simulink model "COMPONENT_MDL_Lag_QUAD_and_PEND_with_spin_rotors"  (R2020b)
(part 10 of 10)

(Lx_pend.^2.*THE_Theta_D.*m_pend.*sin(THE_Theta_pend.*2.0))./2.4e+1-(Ly_pend.^2.*THE_Theta_D.*m_pend.*sin(THE_Theta_pend.*2.0))./2.4e+1-(Lx_pend.^2.*THE_Psi_D.*m_pend.*cos(THE_Phi_pend).*sin(THE_Psi))./6.0-(Ly_pend.^2.*THE_Phi_pend_D.*m_pend.*cos(THE_Psi).*sin(THE_Phi_pend))./6.0-(Ly_pend.^2.*THE_Psi_pend_D.*m_pend.*cos(THE_Theta_pend).*sin(THE_Psi))./6.0-(Lx_pend.^2.*THE_Theta_D.*m_pend.*cos(THE_Psi).*sin(THE_Psi).*sin(THE_Phi_pend))./1.2e+1-(Lx_pend.^2.*THE_Phi_pend_D.*m_pend.*cos(THE_Theta_pend).*sin(THE_Psi).*sin(THE_Theta_pend))./6.0+(Ly_pend.^2.*THE_Theta_D.*m_pend.*cos(THE_Psi).*sin(THE_Psi).*sin(THE_Phi_pend))./1.2e+1+(Ly_pend.^2.*THE_Psi_pend_D.*m_pend.*cos(THE_Psi).*sin(THE_Phi_pend).*sin(THE_Theta_pend))./6.0+(Ly_pend.^2.*THE_Phi_pend_D.*m_pend.*cos(THE_Theta_pend).*sin(THE_Psi).*sin(THE_Theta_pend))./6.0+(Lx_pend.^2.*THE_Psi_D.*m_pend.*cos(THE_Phi_pend).*cos(THE_Theta_pend).^2.*sin(THE_Psi))./6.0-(Lx_pend.^2.*THE_Theta_D.*m_pend.*cos(THE_Psi).^2.*cos(THE_Theta_pend).*sin(THE_Theta_pend))./6.0-(Lx_pend.^2.*THE_Phi_pend_D.*m_pend.*cos(THE_Psi).*cos(THE_Theta_pend).^2.*sin(THE_Phi_pend))./6.0-(Ly_pend.^2.*THE_Psi_D.*m_pend.*cos(THE_Phi_pend).*cos(THE_Theta_pend).^2.*sin(THE_Psi))./6.0+(Ly_pend.^2.*THE_Phi_pend_D.*m_pend.*cos(THE_Psi).*cos(THE_Psi_pend).^2.*sin(THE_Phi_pend))./6.0+(Ly_pend.^2.*THE_Theta_D.*m_pend.*cos(THE_Psi).^2.*cos(THE_Theta_pend).*sin(THE_Theta_pend))./6.0+(Ly_pend.^2.*THE_Phi_pend_D.*m_pend.*cos(THE_Psi).*cos(THE_Theta_pend).^2.*sin(THE_Phi_pend))./6.0+(Ly_pend.^2.*THE_Psi_pend_D.*m_pend.*cos(THE_Psi_pend).^2.*cos(THE_Theta_pend).*sin(THE_Psi))./6.0+(Ly_pend.^2.*THE_Theta_D.*m_pend.*cos(THE_Psi_pend).^2.*cos(THE_Theta_pend).*sin(THE_Theta_pend))./1.2e+1-Lz_pend.^2.*THE_Phi_pend_D.*m_pend.*cos(THE_Psi).*cos(THE_Psi_pend).^2.*sin(THE_Phi_pend).*(2.0./3.0)-Lz_pend.^2.*THE_Psi_pend_D.*m_pend.*cos(THE_Psi_pend).^2.*cos(THE_Theta_pend).*sin(THE_Psi).*(2.0./3.0)-(Lz_pend.^2.*THE_Theta_D.*m_pend.*cos(THE_Psi_pend).^2.*cos(THE_Theta_pend).*sin(THE_Theta_pend))./3.0+(Lx_pend.^2.*THE_Theta_D.*m_pend.*cos(THE_Psi).*cos(THE_Theta_pend).^2.*sin(THE_Psi).*sin(THE_Phi_pend))./6.0-(Ly_pend.^2.*THE_Theta_D.*m_pend.*cos(THE_Psi).*cos(THE_Psi_pend).^2.*sin(THE_Psi).*sin(THE_Phi_pend))./1.2e+1-(Ly_pend.^2.*THE_Theta_D.*m_pend.*cos(THE_Psi).*cos(THE_Theta_pend).^2.*sin(THE_Psi).*sin(THE_Phi_pend))./6.0-(Ly_pend.^2.*THE_Psi_pend_D.*m_pend.*cos(THE_Psi).*cos(THE_Psi_pend).^2.*sin(THE_Phi_pend).*sin(THE_Theta_pend))./6.0-(Ly_pend.^2.*THE_Phi_pend_D.*m_pend.*cos(THE_Psi_pend).^2.*cos(THE_Theta_pend).*sin(THE_Psi).*sin(THE_Theta_pend))./6.0+(Lz_pend.^2.*THE_Theta_D.*m_pend.*cos(THE_Psi).*cos(THE_Psi_pend).^2.*sin(THE_Psi).*sin(THE_Phi_pend))./3.0+Lz_pend.^2.*THE_Psi_pend_D.*m_pend.*cos(THE_Psi).*cos(THE_Psi_pend).^2.*sin(THE_Phi_pend).*sin(THE_Theta_pend).*(2.0./3.0)+Lz_pend.^2.*THE_Phi_pend_D.*m_pend.*cos(THE_Psi_pend).^2.*cos(THE_Theta_pend).*sin(THE_Psi).*sin(THE_Theta_pend).*(2.0./3.0)+(Lz_pend.*THE_Theta_D.*Tv_Z_pend.*m_pend.*cos(THE_Psi).^2.*cos(THE_Psi_pend).*sin(THE_Theta_pend))./2.0+(Lx_pend.^2.*THE_Theta_D.*m_pend.*cos(THE_Psi).^2.*cos(THE_Phi_pend).^2.*cos(THE_Theta_pend).*sin(THE_Theta_pend))./1.2e+1+(Ly_pend.^2.*THE_Psi_D.*m_pend.*cos(THE_Phi_pend).*cos(THE_Psi_pend).^2.*cos(THE_Theta_pend).^2.*sin(THE_Psi))./6.0-(Ly_pend.^2.*THE_Theta_D.*m_pend.*cos(THE_Psi).^2.*cos(THE_Phi_pend).^2.*cos(THE_Theta_pend).*sin(THE_Theta_pend))./1.2e+1-(Ly_pend.^2.*THE_Theta_D.*m_pend.*cos(THE_Psi).^2.*cos(THE_Psi_pend).^2.*cos(THE_Theta_pend).*sin(THE_Theta_pend))./6.0-(Ly_pend.^2.*THE_Phi_pend_D.*m_pend.*cos(THE_Psi).*cos(THE_Psi_pend).^2.*cos(THE_Theta_pend).^2.*sin(THE_Phi_pend))./6.0-Lz_pend.^2.*THE_Psi_D.*m_pend.*cos(THE_Phi_pend).*cos(THE_Psi_pend).^2.*cos(THE_Theta_pend).^2.*sin(THE_Psi).*(2.0./3.0)+Lz_pend.^2.*THE_Theta_D.*m_pend.*cos(THE_Psi).^2.*cos(THE_Psi_pend).^2.*cos(THE_Theta_pend).*sin(THE_Theta_pend).*(2.0./3.0)+Lz_pend.^2.*THE_Phi_pend_D.*m_pend.*cos(THE_Psi).*cos(THE_Psi_pend).^2.*cos(THE_Theta_pend).^2.*sin(THE_Phi_pend).*(2.0./3.0)+(Ly_pend.^2.*THE_Psi_pend_D.*m_pend.*cos(THE_Psi).*cos(THE_Phi_pend).*cos(THE_Psi_pend).*sin(THE_Psi_pend))./6.0-Lz_pend.^2.*THE_Psi_pend_D.*m_pend.*cos(THE_Psi).*cos(THE_Phi_pend).*cos(THE_Psi_pend).*sin(THE_Psi_pend).*(2.0./3.0)+(Ly_pend.^2.*THE_Theta_D.*m_pend.*cos(THE_Psi).*cos(THE_Psi_pend).^2.*cos(THE_Theta_pend).^2.*sin(THE_Psi).*sin(THE_Phi_pend))./6.0-Lz_pend.^2.*THE_Theta_D.*m_pend.*cos(THE_Psi).*cos(THE_Psi_pend).^2.*cos(THE_Theta_pend).^2.*sin(THE_Psi).*sin(THE_Phi_pend).*(2.0./3.0)-(Lx_pend.^2.*THE_Psi_D.*m_pend.*cos(THE_Psi).*cos(THE_Phi_pend).*cos(THE_Theta_pend).*sin(THE_Phi_pend).*sin(THE_Theta_pend))./6.0+(Ly_pend.^2.*THE_Psi_D.*m_pend.*cos(THE_Psi).*cos(THE_Phi_pend).*cos(THE_Theta_pend).*sin(THE_Phi_pend).*sin(THE_Theta_pend))./6.0-(Ly_pend.^2.*THE_Phi_pend_D.*m_pend.*cos(THE_Psi).*cos(THE_Phi_pend).*cos(THE_Psi_pend).*sin(THE_Psi_pend).*sin(THE_Theta_pend))./6.0+Lz_pend.^2.*THE_Phi_pend_D.*m_pend.*cos(THE_Psi).*cos(THE_Phi_pend).*cos(THE_Psi_pend).*sin(THE_Psi_pend).*sin(THE_Theta_pend).*(2.0./3.0)+(Ly_pend.^2.*THE_Theta_D.*m_pend.*cos(THE_Psi).^2.*cos(THE_Phi_pend).^2.*cos(THE_Psi_pend).^2.*cos(THE_Theta_pend).*sin(THE_Theta_pend))./1.2e+1-(Lz_pend.^2.*THE_Theta_D.*m_pend.*cos(THE_Psi).^2.*cos(THE_Phi_pend).^2.*cos(THE_Psi_pend).^2.*cos(THE_Theta_pend).*sin(THE_Theta_pend))./3.0-Lz_pend.*THE_Psi_D.*Tv_Z_pend.*m_pend.*cos(THE_Phi_pend).*cos(THE_Psi_pend).*cos(THE_Theta_pend).*sin(THE_Psi)+(Ly_pend.^2.*THE_Psi_D.*m_pend.*cos(THE_Psi).*cos(THE_Phi_pend).^2.*cos(THE_Psi_pend).*cos(THE_Theta_pend).*sin(THE_Psi_pend))./6.0-Lz_pend.^2.*THE_Psi_D.*m_pend.*cos(THE_Psi).*cos(THE_Phi_pend).^2.*cos(THE_Psi_pend).*cos(THE_Theta_pend).*sin(THE_Psi_pend).*(2.0./3.0)+(Ly_pend.^2.*THE_Theta_D.*m_pend.*cos(THE_Psi).*cos(THE_Phi_pend).*cos(THE_Psi_pend).*sin(THE_Psi).*sin(THE_Psi_pend).*sin(THE_Theta_pend))./1.2e+1-(Lz_pend.^2.*THE_Theta_D.*m_pend.*cos(THE_Psi).*cos(THE_Phi_pend).*cos(THE_Psi_pend).*sin(THE_Psi).*sin(THE_Psi_pend).*sin(THE_Theta_pend))./3.0-(Lz_pend.*THE_Theta_D.*Tv_Z_pend.*m_pend.*cos(THE_Psi).*cos(THE_Psi_pend).*cos(THE_Theta_pend).*sin(THE_Psi).*sin(THE_Phi_pend))./2.0-(Ly_pend.^2.*THE_Psi_D.*m_pend.*cos(THE_Psi).*cos(THE_Phi_pend).*cos(THE_Psi_pend).^2.*cos(THE_Theta_pend).*sin(THE_Phi_pend).*sin(THE_Theta_pend))./6.0+(Ly_pend.^2.*THE_Theta_D.*m_pend.*cos(THE_Psi).^2.*cos(THE_Phi_pend).*cos(THE_Psi_pend).*cos(THE_Theta_pend).*sin(THE_Phi_pend).*sin(THE_Psi_pend))./1.2e+1+Lz_pend.^2.*THE_Psi_D.*m_pend.*cos(THE_Psi).*cos(THE_Phi_pend).*cos(THE_Psi_pend).^2.*cos(THE_Theta_pend).*sin(THE_Phi_pend).*sin(THE_Theta_pend).*(2.0./3.0)-(Lz_pend.^2.*THE_Theta_D.*m_pend.*cos(THE_Psi).^2.*cos(THE_Phi_pend).*cos(THE_Psi_pend).*cos(THE_Theta_pend).*sin(THE_Phi_pend).*sin(THE_Psi_pend))./3.0,(Ly_pend.^2.*THE_Psi_D.*m_pend.*cos(THE_Psi).*sin(THE_Theta_pend))./6.0+(Ly_pend.^2.*THE_Theta_pend_D.*m_pend.*cos(THE_Theta_pend).*sin(THE_Psi))./6.0-(Ly_pend.^2.*THE_Psi_D.*m_pend.*cos(THE_Theta_pend).*sin(THE_Psi).*sin(THE_Phi_pend))./6.0-(Ly_pend.^2.*THE_Theta_pend_D.*m_pend.*cos(THE_Psi).*sin(THE_Phi_pend).*sin(THE_Theta_pend))./6.0-(Ly_pend.^2.*THE_Psi_D.*m_pend.*cos(THE_Psi).*cos(THE_Phi_pend).^2.*sin(THE_Theta_pend))./6.0-(Ly_pend.^2.*THE_Psi_D.*m_pend.*cos(THE_Psi).*cos(THE_Psi_pend).^2.*sin(THE_Theta_pend))./6.0+(Ly_pend.^2.*THE_Theta_D.*m_pend.*cos(THE_Psi).^2.*cos(THE_Psi_pend).*sin(THE_Psi_pend))./1.2e+1+(Ly_pend.^2.*THE_Theta_D.*m_pend.*cos(THE_Psi_pend).*cos(THE_Theta_pend).^2.*sin(THE_Psi_pend))./1.2e+1-(Ly_pend.^2.*THE_Theta_pend_D.*m_pend.*cos(THE_Psi_pend).^2.*cos(THE_Theta_pend).*sin(THE_Psi))./6.0+Lz_pend.^2.*THE_Psi_D.*m_pend.*cos(THE_Psi).*cos(THE_Phi_pend).^2.*sin(THE_Theta_pend).*(2.0./3.0)+Lz_pend.^2.*THE_Psi_D.*m_pend.*cos(THE_Psi).*cos(THE_Psi_pend).^2.*sin(THE_Theta_pend).*(2.0./3.0)-(Lz_pend.^2.*THE_Theta_D.*m_pend.*cos(THE_Psi).^2.*cos(THE_Psi_pend).*sin(THE_Psi_pend))./3.0-(Lz_pend.^2.*THE_Theta_D.*m_pend.*cos(THE_Psi_pend).*cos(THE_Theta_pend).^2.*sin(THE_Psi_pend))./3.0+Lz_pend.^2.*THE_Theta_pend_D.*m_pend.*cos(THE_Psi_pend).^2.*cos(THE_Theta_pend).*sin(THE_Psi).*(2.0./3.0)+Lz_pend.^2.*THE_Phi_pend_D.*m_pend.*cos(THE_Psi).*cos(THE_Phi_pend).*cos(THE_Theta_pend).*(2.0./3.0)-Lz_pend.*THE_Psi_D.*Tv_Z_pend.*m_pend.*cos(THE_Psi_pend).*sin(THE_Psi).*sin(THE_Phi_pend)+(Ly_pend.^2.*THE_Phi_pend_D.*m_pend.*cos(THE_Psi).*cos(THE_Phi_pend).*cos(THE_Psi_pend).^2.*cos(THE_Theta_pend))./6.0-Lz_pend.^2.*THE_Phi_pend_D.*m_pend.*cos(THE_Psi).*cos(THE_Phi_pend).*cos(THE_Psi_pend).^2.*cos(THE_Theta_pend).*(2.0./3.0)+(Ly_pend.^2.*THE_Psi_D.*m_pend.*cos(THE_Psi_pend).^2.*cos(THE_Theta_pend).*sin(THE_Psi).*sin(THE_Phi_pend))./6.0-(Ly_pend.^2.*THE_Theta_D.*m_pend.*cos(THE_Psi).^2.*cos(THE_Phi_pend).*sin(THE_Phi_pend).*sin(THE_Theta_pend))./1.2e+1-(Ly_pend.^2.*THE_Phi_pend_D.*m_pend.*cos(THE_Psi_pend).*cos(THE_Theta_pend).^2.*sin(THE_Psi).*sin(THE_Psi_pend))./6.0+(Ly_pend.^2.*THE_Theta_pend_D.*m_pend.*cos(THE_Psi).*cos(THE_Psi_pend).^2.*sin(THE_Phi_pend).*sin(THE_Theta_pend))./6.0-Lz_pend.^2.*THE_Psi_D.*m_pend.*cos(THE_Psi_pend).^2.*cos(THE_Theta_pend).*sin(THE_Psi).*sin(THE_Phi_pend).*(2.0./3.0)+(Lz_pend.^2.*THE_Theta_D.*m_pend.*cos(THE_Psi).^2.*cos(THE_Phi_pend).*sin(THE_Phi_pend).*sin(THE_Theta_pend))./3.0+Lz_pend.^2.*THE_Phi_pend_D.*m_pend.*cos(THE_Psi_pend).*cos(THE_Theta_pend).^2.*sin(THE_Psi).*sin(THE_Psi_pend).*(2.0./3.0)-Lz_pend.^2.*THE_Theta_pend_D.*m_pend.*cos(THE_Psi).*cos(THE_Psi_pend).^2.*sin(THE_Phi_pend).*sin(THE_Theta_pend).*(2.0./3.0)+(Lz_pend.*THE_Theta_D.*Tv_Z_pend.*m_pend.*cos(THE_Psi).^2.*cos(THE_Theta_pend).*sin(THE_Psi_pend))./2.0+(Ly_pend.^2.*THE_Psi_D.*m_pend.*cos(THE_Psi).*cos(THE_Phi_pend).^2.*cos(THE_Psi_pend).^2.*sin(THE_Theta_pend))./3.0-(Ly_pend.^2.*THE_Theta_D.*m_pend.*cos(THE_Psi).^2.*cos(THE_Phi_pend).^2.*cos(THE_Psi_pend).*sin(THE_Psi_pend))./6.0-(Ly_pend.^2.*THE_Theta_D.*m_pend.*cos(THE_Psi).^2.*cos(THE_Psi_pend).*cos(THE_Theta_pend).^2.*sin(THE_Psi_pend))./6.0-Lz_pend.^2.*THE_Psi_D.*m_pend.*cos(THE_Psi).*cos(THE_Phi_pend).^2.*cos(THE_Psi_pend).^2.*sin(THE_Theta_pend).*(4.0./3.0)+Lz_pend.^2.*THE_Theta_D.*m_pend.*cos(THE_Psi).^2.*cos(THE_Phi_pend).^2.*cos(THE_Psi_pend).*sin(THE_Psi_pend).*(2.0./3.0)+Lz_pend.^2.*THE_Theta_D.*m_pend.*cos(THE_Psi).^2.*cos(THE_Psi_pend).*cos(THE_Theta_pend).^2.*sin(THE_Psi_pend).*(2.0./3.0)+(Ly_pend.^2.*THE_Theta_D.*m_pend.*cos(THE_Psi).*cos(THE_Phi_pend).*cos(THE_Theta_pend).*sin(THE_Psi))./1.2e+1-(Ly_pend.^2.*THE_Theta_pend_D.*m_pend.*cos(THE_Psi).*cos(THE_Phi_pend).*cos(THE_Psi_pend).*sin(THE_Psi_pend))./6.0-(Lz_pend.^2.*THE_Theta_D.*m_pend.*cos(THE_Psi).*cos(THE_Phi_pend).*cos(THE_Theta_pend).*sin(THE_Psi))./3.0+Lz_pend.^2.*THE_Theta_pend_D.*m_pend.*cos(THE_Psi).*cos(THE_Phi_pend).*cos(THE_Psi_pend).*sin(THE_Psi_pend).*(2.0./3.0)+(Ly_pend.^2.*THE_Theta_D.*m_pend.*cos(THE_Psi).^2.*cos(THE_Phi_pend).*cos(THE_Psi_pend).^2.*sin(THE_Phi_pend).*sin(THE_Theta_pend))./6.0-Lz_pend.^2.*THE_Theta_D.*m_pend.*cos(THE_Psi).^2.*cos(THE_Phi_pend).*cos(THE_Psi_pend).^2.*sin(THE_Phi_pend).*sin(THE_Theta_pend).*(2.0./3.0)+(Ly_pend.^2.*THE_Psi_D.*m_pend.*cos(THE_Psi).*cos(THE_Phi_pend).*cos(THE_Psi_pend).*sin(THE_Phi_pend).*sin(THE_Psi_pend))./3.0-Lz_pend.^2.*THE_Psi_D.*m_pend.*cos(THE_Psi).*cos(THE_Phi_pend).*cos(THE_Psi_pend).*sin(THE_Phi_pend).*sin(THE_Psi_pend).*(4.0./3.0)+(Ly_pend.^2.*THE_Theta_D.*m_pend.*cos(THE_Psi).^2.*cos(THE_Phi_pend).^2.*cos(THE_Psi_pend).*cos(THE_Theta_pend).^2.*sin(THE_Psi_pend))./1.2e+1-(Lz_pend.^2.*THE_Theta_D.*m_pend.*cos(THE_Psi).^2.*cos(THE_Phi_pend).^2.*cos(THE_Psi_pend).*cos(THE_Theta_pend).^2.*sin(THE_Psi_pend))./3.0+(Lz_pend.*THE_Theta_D.*Tv_Z_pend.*m_pend.*cos(THE_Psi).*cos(THE_Phi_pend).*cos(THE_Psi_pend).*sin(THE_Psi))./2.0+Lz_pend.*THE_Psi_D.*Tv_Z_pend.*m_pend.*cos(THE_Phi_pend).*sin(THE_Psi).*sin(THE_Psi_pend).*sin(THE_Theta_pend)-(Ly_pend.^2.*THE_Theta_D.*m_pend.*cos(THE_Psi).*cos(THE_Phi_pend).*cos(THE_Psi_pend).^2.*cos(THE_Theta_pend).*sin(THE_Psi))./6.0+Lz_pend.^2.*THE_Theta_D.*m_pend.*cos(THE_Psi).*cos(THE_Phi_pend).*cos(THE_Psi_pend).^2.*cos(THE_Theta_pend).*sin(THE_Psi).*(2.0./3.0)-(Ly_pend.^2.*THE_Psi_D.*m_pend.*cos(THE_Phi_pend).*cos(THE_Psi_pend).*cos(THE_Theta_pend).*sin(THE_Psi).*sin(THE_Psi_pend).*sin(THE_Theta_pend))./6.0+(Ly_pend.^2.*THE_Phi_pend_D.*m_pend.*cos(THE_Psi).*cos(THE_Psi_pend).*cos(THE_Theta_pend).*sin(THE_Phi_pend).*sin(THE_Psi_pend).*sin(THE_Theta_pend))./6.0+Lz_pend.^2.*THE_Psi_D.*m_pend.*cos(THE_Phi_pend).*cos(THE_Psi_pend).*cos(THE_Theta_pend).*sin(THE_Psi).*sin(THE_Psi_pend).*sin(THE_Theta_pend).*(2.0./3.0)-Lz_pend.^2.*THE_Phi_pend_D.*m_pend.*cos(THE_Psi).*cos(THE_Psi_pend).*cos(THE_Theta_pend).*sin(THE_Phi_pend).*sin(THE_Psi_pend).*sin(THE_Theta_pend).*(2.0./3.0)+(Lz_pend.*THE_Theta_D.*Tv_Z_pend.*m_pend.*cos(THE_Psi).*sin(THE_Psi).*sin(THE_Phi_pend).*sin(THE_Psi_pend).*sin(THE_Theta_pend))./2.0-(Ly_pend.^2.*THE_Psi_D.*m_pend.*cos(THE_Psi).*cos(THE_Phi_pend).*cos(THE_Psi_pend).*cos(THE_Theta_pend).^2.*sin(THE_Phi_pend).*sin(THE_Psi_pend))./6.0+Lz_pend.^2.*THE_Psi_D.*m_pend.*cos(THE_Psi).*cos(THE_Phi_pend).*cos(THE_Psi_pend).*cos(THE_Theta_pend).^2.*sin(THE_Phi_pend).*sin(THE_Psi_pend).*(2.0./3.0)-(Ly_pend.^2.*THE_Theta_D.*m_pend.*cos(THE_Psi).*cos(THE_Psi_pend).*cos(THE_Theta_pend).*sin(THE_Psi).*sin(THE_Phi_pend).*sin(THE_Psi_pend).*sin(THE_Theta_pend))./6.0+Lz_pend.^2.*THE_Theta_D.*m_pend.*cos(THE_Psi).*cos(THE_Psi_pend).*cos(THE_Theta_pend).*sin(THE_Psi).*sin(THE_Phi_pend).*sin(THE_Psi_pend).*sin(THE_Theta_pend).*(2.0./3.0),I_xy.*THE_Psi_D.*cos(THE_Psi).*cos(THE_Theta)+Iprop_xy.*THE_Psi_D.*cos(THE_Psi).*cos(THE_Theta).*4.0-I_xz.*THE_Psi_D.*cos(THE_Theta).*sin(THE_Psi)-Iprop_xz.*THE_Psi_D.*cos(THE_Theta).*sin(THE_Psi).*4.0+Iprop_yz.*wMOT_1.*cos(THE_Psi).*cos(THE_Theta)+Iprop_yz.*wMOT_2.*cos(THE_Psi).*cos(THE_Theta)+Iprop_yz.*wMOT_3.*cos(THE_Psi).*cos(THE_Theta)+Iprop_yz.*wMOT_4.*cos(THE_Psi).*cos(THE_Theta)-Iprop_zz.*wMOT_1.*cos(THE_Theta).*sin(THE_Psi)-Iprop_zz.*wMOT_2.*cos(THE_Theta).*sin(THE_Psi)-Iprop_zz.*wMOT_3.*cos(THE_Theta).*sin(THE_Psi)-Iprop_zz.*wMOT_4.*cos(THE_Theta).*sin(THE_Psi)-Lz_pend.^2.*THE_Phi_pend_D.*m_pend.*cos(THE_Theta).*sin(THE_Psi).*(2.0./3.0)-(Ly_pend.^2.*THE_Phi_pend_D.*m_pend.*cos(THE_Phi_pend).*sin(THE_Theta).*sin(THE_Phi_pend))./6.0-(Ly_pend.^2.*THE_Psi_pend_D.*m_pend.*cos(THE_Psi_pend).*sin(THE_Theta).*sin(THE_Psi_pend))./6.0+Lz_pend.^2.*THE_Psi_pend_D.*m_pend.*cos(THE_Theta).*sin(THE_Psi).*sin(THE_Theta_pend).*(2.0./3.0)+Lz_pend.^2.*THE_Phi_pend_D.*m_pend.*cos(THE_Phi_pend).*sin(THE_Theta).*sin(THE_Phi_pend).*(2.0./3.0)+Lz_pend.^2.*THE_Psi_pend_D.*m_pend.*cos(THE_Psi_pend).*sin(THE_Theta).*sin(THE_Psi_pend).*(2.0./3.0)-(Ly_pend.^2.*THE_Phi_pend_D.*m_pend.*cos(THE_Theta).*cos(THE_Phi_pend).^2.*sin(THE_Psi))./6.0-(Ly_pend.^2.*THE_Phi_pend_D.*m_pend.*cos(THE_Theta).*cos(THE_Psi_pend).^2.*sin(THE_Psi))./6.0+Lz_pend.^2.*THE_Phi_pend_D.*m_pend.*cos(THE_Theta).*cos(THE_Phi_pend).^2.*sin(THE_Psi).*(2.0./3.0)+Lz_pend.^2.*THE_Phi_pend_D.*m_pend.*cos(THE_Theta).*cos(THE_Psi_pend).^2.*sin(THE_Psi).*(2.0./3.0)+(Ly_pend.^2.*THE_Theta_pend_D.*m_pend.*cos(THE_Psi).*cos(THE_Theta).*cos(THE_Phi_pend))./6.0+Lz_pend.*THE_Psi_pend_D.*Tv_Z_pend.*m_pend.*cos(THE_Theta_pend).*sin(THE_Theta).*sin(THE_Psi_pend)+Lz_pend.*THE_Theta_pend_D.*Tv_Z_pend.*m_pend.*cos(THE_Psi_pend).*sin(THE_Theta).*sin(THE_Theta_pend)+(Lx_pend.^2.*THE_Theta_pend_D.*m_pend.*cos(THE_Psi).*cos(THE_Theta).*cos(THE_Phi_pend).*cos(THE_Theta_pend).^2)./6.0-(Ly_pend.^2.*THE_Theta_pend_D.*m_pend.*cos(THE_Psi).*cos(THE_Theta).*cos(THE_Phi_pend).*cos(THE_Psi_pend).^2)./6.0-(Ly_pend.^2.*THE_Theta_pend_D.*m_pend.*cos(THE_Psi).*cos(THE_Theta).*cos(THE_Phi_pend).*cos(THE_Theta_pend).^2)./6.0+Lz_pend.^2.*THE_Theta_pend_D.*m_pend.*cos(THE_Psi).*cos(THE_Theta).*cos(THE_Phi_pend).*cos(THE_Psi_pend).^2.*(2.0./3.0)-(Lx_pend.^2.*THE_Phi_pend_D.*m_pend.*cos(THE_Phi_pend).*cos(THE_Theta_pend).^2.*sin(THE_Theta).*sin(THE_Phi_pend))./6.0-(Lx_pend.^2.*THE_Theta_pend_D.*m_pend.*cos(THE_Phi_pend).^2.*cos(THE_Theta_pend).*sin(THE_Theta).*sin(THE_Theta_pend))./6.0+(Ly_pend.^2.*THE_Psi_pend_D.*m_pend.*cos(THE_Theta).*cos(THE_Phi_pend).^2.*sin(THE_Psi).*sin(THE_Theta_pend))./6.0+(Ly_pend.^2.*THE_Psi_pend_D.*m_pend.*cos(THE_Theta).*cos(THE_Psi_pend).^2.*sin(THE_Psi).*sin(THE_Theta_pend))./6.0+(Ly_pend.^2.*THE_Phi_pend_D.*m_pend.*cos(THE_Phi_pend).*cos(THE_Psi_pend).^2.*sin(THE_Theta).*sin(THE_Phi_pend))./3.0+(Ly_pend.^2.*THE_Psi_pend_D.*m_pend.*cos(THE_Phi_pend).^2.*cos(THE_Psi_pend).*sin(THE_Theta).*sin(THE_Psi_pend))./3.0+(Ly_pend.^2.*THE_Phi_pend_D.*m_pend.*cos(THE_Phi_pend).*cos(THE_Theta_pend).^2.*sin(THE_Theta).*sin(THE_Phi_pend))./6.0+(Ly_pend.^2.*THE_Theta_pend_D.*m_pend.*cos(THE_Phi_pend).^2.*cos(THE_Theta_pend).*sin(THE_Theta).*sin(THE_Theta_pend))./6.0-Lz_pend.^2.*THE_Psi_pend_D.*m_pend.*cos(THE_Theta).*cos(THE_Phi_pend).^2.*sin(THE_Psi).*sin(THE_Theta_pend).*(2.0./3.0)-Lz_pend.^2.*THE_Psi_pend_D.*m_pend.*cos(THE_Theta).*cos(THE_Psi_pend).^2.*sin(THE_Psi).*sin(THE_Theta_pend).*(2.0./3.0)-Lz_pend.^2.*THE_Phi_pend_D.*m_pend.*cos(THE_Phi_pend).*cos(THE_Psi_pend).^2.*sin(THE_Theta).*sin(THE_Phi_pend).*(4.0./3.0)-Lz_pend.^2.*THE_Psi_pend_D.*m_pend.*cos(THE_Phi_pend).^2.*cos(THE_Psi_pend).*sin(THE_Theta).*sin(THE_Psi_pend).*(4.0./3.0)-(Lx_pend.^2.*THE_Phi_pend_D.*m_pend.*cos(THE_Theta).*cos(THE_Phi_pend).^2.*cos(THE_Theta_pend).^2.*sin(THE_Psi))./6.0+(Ly_pend.^2.*THE_Phi_pend_D.*m_pend.*cos(THE_Theta).*cos(THE_Phi_pend).^2.*cos(THE_Psi_pend).^2.*sin(THE_Psi))./3.0+(Ly_pend.^2.*THE_Phi_pend_D.*m_pend.*cos(THE_Theta).*cos(THE_Phi_pend).^2.*cos(THE_Theta_pend).^2.*sin(THE_Psi))./6.0-Lz_pend.^2.*THE_Phi_pend_D.*m_pend.*cos(THE_Theta).*cos(THE_Phi_pend).^2.*cos(THE_Psi_pend).^2.*sin(THE_Psi).*(4.0./3.0)-(Ly_pend.^2.*THE_Psi_D.*m_pend.*cos(THE_Psi).*cos(THE_Theta).*cos(THE_Phi_pend).*sin(THE_Phi_pend))./1.2e+1+(Lz_pend.^2.*THE_Psi_D.*m_pend.*cos(THE_Psi).*cos(THE_Theta).*cos(THE_Phi_pend).*sin(THE_Phi_pend))./3.0+Lz_pend.^2.*THE_Psi_pend_D.*m_pend.*cos(THE_Psi).*cos(THE_Theta).*cos(THE_Theta_pend).*sin(THE_Phi_pend).*(2.0./3.0)+(Ly_pend.^2.*THE_Psi_pend_D.*m_pend.*cos(THE_Phi_pend).*sin(THE_Theta).*sin(THE_Phi_pend).*sin(THE_Theta_pend))./6.0+(Ly_pend.^2.*THE_Phi_pend_D.*m_pend.*cos(THE_Psi_pend).*sin(THE_Theta).*sin(THE_Psi_pend).*sin(THE_Theta_pend))./6.0-Lz_pend.^2.*THE_Psi_pend_D.*m_pend.*cos(THE_Phi_pend).*sin(THE_Theta).*sin(THE_Phi_pend).*sin(THE_Theta_pend).*(2.0./3.0)-Lz_pend.^2.*THE_Phi_pend_D.*m_pend.*cos(THE_Psi_pend).*sin(THE_Theta).*sin(THE_Psi_pend).*sin(THE_Theta_pend).*(2.0./3.0)+(Ly_pend.^2.*THE_Theta_pend_D.*m_pend.*cos(THE_Psi).*cos(THE_Theta).*cos(THE_Phi_pend).*cos(THE_Psi_pend).^2.*cos(THE_Theta_pend).^2)./6.0-Lz_pend.^2.*THE_Theta_pend_D.*m_pend.*cos(THE_Psi).*cos(THE_Theta).*cos(THE_Phi_pend).*cos(THE_Psi_pend).^2.*cos(THE_Theta_pend).^2.*(2.0./3.0)-(Ly_pend.^2.*THE_Psi_pend_D.*m_pend.*cos(THE_Theta).*cos(THE_Phi_pend).^2.*cos(THE_Psi_pend).^2.*sin(THE_Psi).*sin(THE_Theta_pend))./3.0-(Ly_pend.^2.*THE_Phi_pend_D.*m_pend.*cos(THE_Phi_pend).*cos(THE_Psi_pend).^2.*cos(THE_Theta_pend).^2.*sin(THE_Theta).*sin(THE_Phi_pend))./6.0-(Ly_pend.^2.*THE_Psi_pend_D.*m_pend.*cos(THE_Phi_pend).^2.*cos(THE_Psi_pend).*cos(THE_Theta_pend).^2.*sin(THE_Theta).*sin(THE_Psi_pend))./6.0-(Ly_pend.^2.*THE_Theta_pend_D.*m_pend.*cos(THE_Phi_pend).^2.*cos(THE_Psi_pend).^2.*cos(THE_Theta_pend).*sin(THE_Theta).*sin(THE_Theta_pend))./6.0+Lz_pend.^2.*THE_Psi_pend_D.*m_pend.*cos(THE_Theta).*cos(THE_Phi_pend).^2.*cos(THE_Psi_pend).^2.*sin(THE_Psi).*sin(THE_Theta_pend).*(4.0./3.0)+Lz_pend.^2.*THE_Phi_pend_D.*m_pend.*cos(THE_Phi_pend).*cos(THE_Psi_pend).^2.*cos(THE_Theta_pend).^2.*sin(THE_Theta).*sin(THE_Phi_pend).*(2.0./3.0)+Lz_pend.^2.*THE_Psi_pend_D.*m_pend.*cos(THE_Phi_pend).^2.*cos(THE_Psi_pend).*cos(THE_Theta_pend).^2.*sin(THE_Theta).*sin(THE_Psi_pend).*(2.0./3.0)+Lz_pend.^2.*THE_Theta_pend_D.*m_pend.*cos(THE_Phi_pend).^2.*cos(THE_Psi_pend).^2.*cos(THE_Theta_pend).*sin(THE_Theta).*sin(THE_Theta_pend).*(2.0./3.0)-(Lx_pend.^2.*THE_Psi_D.*m_pend.*cos(THE_Theta).*cos(THE_Phi_pend).*cos(THE_Theta_pend).*sin(THE_Psi).*sin(THE_Theta_pend))./1.2e+1+(Ly_pend.^2.*THE_Psi_D.*m_pend.*cos(THE_Psi).*cos(THE_Theta).*cos(THE_Psi_pend).*sin(THE_Psi_pend).*sin(THE_Theta_pend))./1.2e+1+(Ly_pend.^2.*THE_Psi_D.*m_pend.*cos(THE_Theta).*cos(THE_Phi_pend).*cos(THE_Theta_pend).*sin(THE_Psi).*sin(THE_Theta_pend))./1.2e+1+(Ly_pend.^2.*THE_Theta_pend_D.*m_pend.*cos(THE_Theta).*cos(THE_Psi_pend).*cos(THE_Theta_pend).*sin(THE_Psi).*sin(THE_Psi_pend))./6.0-(Lz_pend.^2.*THE_Psi_D.*m_pend.*cos(THE_Psi).*cos(THE_Theta).*cos(THE_Psi_pend).*sin(THE_Psi_pend).*sin(THE_Theta_pend))./3.0-Lz_pend.^2.*THE_Theta_pend_D.*m_pend.*cos(THE_Theta).*cos(THE_Psi_pend).*cos(THE_Theta_pend).*sin(THE_Psi).*sin(THE_Psi_pend).*(2.0./3.0)-(Ly_pend.^2.*THE_Phi_pend_D.*m_pend.*cos(THE_Theta).*cos(THE_Phi_pend).^2.*cos(THE_Psi_pend).^2.*cos(THE_Theta_pend).^2.*sin(THE_Psi))./6.0+Lz_pend.^2.*THE_Phi_pend_D.*m_pend.*cos(THE_Theta).*cos(THE_Phi_pend).^2.*cos(THE_Psi_pend).^2.*cos(THE_Theta_pend).^2.*sin(THE_Psi).*(2.0./3.0)+(Lz_pend.*THE_Psi_D.*Tv_Z_pend.*m_pend.*cos(THE_Theta).*sin(THE_Psi).*sin(THE_Phi_pend).*sin(THE_Psi_pend))./2.0-(Lx_pend.^2.*THE_Psi_D.*m_pend.*cos(THE_Psi).*cos(THE_Theta).*cos(THE_Phi_pend).*cos(THE_Theta_pend).^2.*sin(THE_Phi_pend))./1.2e+1+(Ly_pend.^2.*THE_Psi_D.*m_pend.*cos(THE_Psi).*cos(THE_Theta).*cos(THE_Phi_pend).*cos(THE_Psi_pend).^2.*sin(THE_Phi_pend))./6.0+(Ly_pend.^2.*THE_Psi_D.*m_pend.*cos(THE_Psi).*cos(THE_Theta).*cos(THE_Phi_pend).*cos(THE_Theta_pend).^2.*sin(THE_Phi_pend))./1.2e+1+(Ly_pend.^2.*THE_Psi_pend_D.*m_pend.*cos(THE_Psi).*cos(THE_Theta).*cos(THE_Psi_pend).^2.*cos(THE_Theta_pend).*sin(THE_Phi_pend))./6.0-Lz_pend.^2.*THE_Psi_D.*m_pend.*cos(THE_Psi).*cos(THE_Theta).*cos(THE_Phi_pend).*cos(THE_Psi_pend).^2.*sin(THE_Phi_pend).*(2.0./3.0)-Lz_pend.^2.*THE_Psi_pend_D.*m_pend.*cos(THE_Psi).*cos(THE_Theta).*cos(THE_Psi_pend).^2.*cos(THE_Theta_pend).*sin(THE_Phi_pend).*(2.0./3.0)-(Ly_pend.^2.*THE_Phi_pend_D.*m_pend.*cos(THE_Phi_pend).^2.*cos(THE_Psi_pend).*sin(THE_Theta).*sin(THE_Psi_pend).*sin(THE_Theta_pend))./3.0-(Ly_pend.^2.*THE_Psi_pend_D.*m_pend.*cos(THE_Phi_pend).*cos(THE_Psi_pend).^2.*sin(THE_Theta).*sin(THE_Phi_pend).*sin(THE_Theta_pend))./3.0+Lz_pend.^2.*THE_Phi_pend_D.*m_pend.*cos(THE_Phi_pend).^2.*cos(THE_Psi_pend).*sin(THE_Theta).*sin(THE_Psi_pend).*sin(THE_Theta_pend).*(4.0./3.0)+Lz_pend.^2.*THE_Psi_pend_D.*m_pend.*cos(THE_Phi_pend).*cos(THE_Psi_pend).^2.*sin(THE_Theta).*sin(THE_Phi_pend).*sin(THE_Theta_pend).*(4.0./3.0)+(Lx_pend.^2.*THE_Theta_pend_D.*m_pend.*cos(THE_Theta).*cos(THE_Phi_pend).*cos(THE_Theta_pend).*sin(THE_Psi).*sin(THE_Phi_pend).*sin(THE_Theta_pend))./6.0-(Ly_pend.^2.*THE_Psi_D.*m_pend.*cos(THE_Theta).*cos(THE_Psi_pend).*cos(THE_Theta_pend).*sin(THE_Psi).*sin(THE_Phi_pend).*sin(THE_Psi_pend))./1.2e+1-(Ly_pend.^2.*THE_Psi_pend_D.*m_pend.*cos(THE_Theta).*cos(THE_Phi_pend).*cos(THE_Psi_pend).*sin(THE_Psi).*sin(THE_Phi_pend).*sin(THE_Psi_pend))./3.0-(Ly_pend.^2.*THE_Theta_pend_D.*m_pend.*cos(THE_Psi).*cos(THE_Theta).*cos(THE_Psi_pend).*sin(THE_Phi_pend).*sin(THE_Psi_pend).*sin(THE_Theta_pend))./6.0-(Ly_pend.^2.*THE_Theta_pend_D.*m_pend.*cos(THE_Theta).*cos(THE_Phi_pend).*cos(THE_Theta_pend).*sin(THE_Psi).*sin(THE_Phi_pend).*sin(THE_Theta_pend))./6.0-(Ly_pend.^2.*THE_Theta_pend_D.*m_pend.*cos(THE_Phi_pend).*cos(THE_Psi_pend).*cos(THE_Theta_pend).*sin(THE_Theta).*sin(THE_Phi_pend).*sin(THE_Psi_pend))./6.0+(Lz_pend.^2.*THE_Psi_D.*m_pend.*cos(THE_Theta).*cos(THE_Psi_pend).*cos(THE_Theta_pend).*sin(THE_Psi).*sin(THE_Phi_pend).*sin(THE_Psi_pend))./3.0+Lz_pend.^2.*THE_Psi_pend_D.*m_pend.*cos(THE_Theta).*cos(THE_Phi_pend).*cos(THE_Psi_pend).*sin(THE_Psi).*sin(THE_Phi_pend).*sin(THE_Psi_pend).*(4.0./3.0)+Lz_pend.^2.*THE_Theta_pend_D.*m_pend.*cos(THE_Psi).*cos(THE_Theta).*cos(THE_Psi_pend).*sin(THE_Phi_pend).*sin(THE_Psi_pend).*sin(THE_Theta_pend).*(2.0./3.0)+Lz_pend.^2.*THE_Theta_pend_D.*m_pend.*cos(THE_Phi_pend).*cos(THE_Psi_pend).*cos(THE_Theta_pend).*sin(THE_Theta).*sin(THE_Phi_pend).*sin(THE_Psi_pend).*(2.0./3.0)+(Lz_pend.*THE_Psi_D.*Tv_Z_pend.*m_pend.*cos(THE_Theta).*cos(THE_Phi_pend).*cos(THE_Psi_pend).*sin(THE_Psi).*sin(THE_Theta_pend))./2.0-(Ly_pend.^2.*THE_Psi_D.*m_pend.*cos(THE_Psi).*cos(THE_Theta).*cos(THE_Phi_pend).^2.*cos(THE_Psi_pend).*sin(THE_Psi_pend).*sin(THE_Theta_pend))./6.0-(Ly_pend.^2.*THE_Psi_D.*m_pend.*cos(THE_Theta).*cos(THE_Phi_pend).*cos(THE_Psi_pend).^2.*cos(THE_Theta_pend).*sin(THE_Psi).*sin(THE_Theta_pend))./1.2e+1-(Ly_pend.^2.*THE_Theta_pend_D.*m_pend.*cos(THE_Theta).*cos(THE_Phi_pend).^2.*cos(THE_Psi_pend).*cos(THE_Theta_pend).*sin(THE_Psi).*sin(THE_Psi_pend))./6.0+Lz_pend.^2.*THE_Psi_D.*m_pend.*cos(THE_Psi).*cos(THE_Theta).*cos(THE_Phi_pend).^2.*cos(THE_Psi_pend).*sin(THE_Psi_pend).*sin(THE_Theta_pend).*(2.0./3.0)+(Lz_pend.^2.*THE_Psi_D.*m_pend.*cos(THE_Theta).*cos(THE_Phi_pend).*cos(THE_Psi_pend).^2.*cos(THE_Theta_pend).*sin(THE_Psi).*sin(THE_Theta_pend))./3.0+Lz_pend.^2.*THE_Theta_pend_D.*m_pend.*cos(THE_Theta).*cos(THE_Phi_pend).^2.*cos(THE_Psi_pend).*cos(THE_Theta_pend).*sin(THE_Psi).*sin(THE_Psi_pend).*(2.0./3.0)-(Ly_pend.^2.*THE_Psi_D.*m_pend.*cos(THE_Psi).*cos(THE_Theta).*cos(THE_Phi_pend).*cos(THE_Psi_pend).^2.*cos(THE_Theta_pend).^2.*sin(THE_Phi_pend))./1.2e+1+(Lz_pend.^2.*THE_Psi_D.*m_pend.*cos(THE_Psi).*cos(THE_Theta).*cos(THE_Phi_pend).*cos(THE_Psi_pend).^2.*cos(THE_Theta_pend).^2.*sin(THE_Phi_pend))./3.0+(Ly_pend.^2.*THE_Phi_pend_D.*m_pend.*cos(THE_Theta).*cos(THE_Phi_pend).*cos(THE_Psi_pend).*sin(THE_Psi).*sin(THE_Phi_pend).*sin(THE_Psi_pend).*sin(THE_Theta_pend))./3.0-Lz_pend.^2.*THE_Phi_pend_D.*m_pend.*cos(THE_Theta).*cos(THE_Phi_pend).*cos(THE_Psi_pend).*sin(THE_Psi).*sin(THE_Phi_pend).*sin(THE_Psi_pend).*sin(THE_Theta_pend).*(4.0./3.0)+(Ly_pend.^2.*THE_Psi_pend_D.*m_pend.*cos(THE_Theta).*cos(THE_Phi_pend).*cos(THE_Psi_pend).*cos(THE_Theta_pend).^2.*sin(THE_Psi).*sin(THE_Phi_pend).*sin(THE_Psi_pend))./6.0+(Ly_pend.^2.*THE_Theta_pend_D.*m_pend.*cos(THE_Theta).*cos(THE_Phi_pend).*cos(THE_Psi_pend).^2.*cos(THE_Theta_pend).*sin(THE_Psi).*sin(THE_Phi_pend).*sin(THE_Theta_pend))./6.0-Lz_pend.^2.*THE_Psi_pend_D.*m_pend.*cos(THE_Theta).*cos(THE_Phi_pend).*cos(THE_Psi_pend).*cos(THE_Theta_pend).^2.*sin(THE_Psi).*sin(THE_Phi_pend).*sin(THE_Psi_pend).*(2.0./3.0)-Lz_pend.^2.*THE_Theta_pend_D.*m_pend.*cos(THE_Theta).*cos(THE_Phi_pend).*cos(THE_Psi_pend).^2.*cos(THE_Theta_pend).*sin(THE_Psi).*sin(THE_Phi_pend).*sin(THE_Theta_pend).*(2.0./3.0)-(Ly_pend.^2.*THE_Psi_pend_D.*m_pend.*cos(THE_Psi).*cos(THE_Theta).*cos(THE_Phi_pend).*cos(THE_Psi_pend).*cos(THE_Theta_pend).*sin(THE_Psi_pend).*sin(THE_Theta_pend))./6.0+Lz_pend.^2.*THE_Psi_pend_D.*m_pend.*cos(THE_Psi).*cos(THE_Theta).*cos(THE_Phi_pend).*cos(THE_Psi_pend).*cos(THE_Theta_pend).*sin(THE_Psi_pend).*sin(THE_Theta_pend).*(2.0./3.0),-I_xz.*THE_Psi_D.*cos(THE_Psi)-Iprop_xz.*THE_Psi_D.*cos(THE_Psi).*4.0-I_xy.*THE_Psi_D.*sin(THE_Psi)-Iprop_xy.*THE_Psi_D.*sin(THE_Psi).*4.0-Iprop_zz.*wMOT_1.*cos(THE_Psi)-Iprop_zz.*wMOT_2.*cos(THE_Psi)-Iprop_zz.*wMOT_3.*cos(THE_Psi)-Iprop_zz.*wMOT_4.*cos(THE_Psi)-Iprop_yz.*wMOT_1.*sin(THE_Psi)-Iprop_yz.*wMOT_2.*sin(THE_Psi)-Iprop_yz.*wMOT_3.*sin(THE_Psi)-Iprop_yz.*wMOT_4.*sin(THE_Psi)-Lz_pend.^2.*THE_Phi_pend_D.*m_pend.*cos(THE_Psi).*(2.0./3.0)-(Ly_pend.^2.*THE_Theta_pend_D.*m_pend.*cos(THE_Phi_pend).*sin(THE_Psi))./6.0+Lz_pend.^2.*THE_Psi_pend_D.*m_pend.*cos(THE_Psi).*sin(THE_Theta_pend).*(2.0./3.0)-(Ly_pend.^2.*THE_Phi_pend_D.*m_pend.*cos(THE_Psi).*cos(THE_Phi_pend).^2)./6.0-(Ly_pend.^2.*THE_Phi_pend_D.*m_pend.*cos(THE_Psi).*cos(THE_Psi_pend).^2)./6.0+Lz_pend.^2.*THE_Phi_pend_D.*m_pend.*cos(THE_Psi).*cos(THE_Phi_pend).^2.*(2.0./3.0)+Lz_pend.^2.*THE_Phi_pend_D.*m_pend.*cos(THE_Psi).*cos(THE_Psi_pend).^2.*(2.0./3.0)+(Ly_pend.^2.*THE_Psi_D.*m_pend.*cos(THE_Phi_pend).*sin(THE_Psi).*sin(THE_Phi_pend))./1.2e+1-(Lz_pend.^2.*THE_Psi_D.*m_pend.*cos(THE_Phi_pend).*sin(THE_Psi).*sin(THE_Phi_pend))./3.0-Lz_pend.^2.*THE_Psi_pend_D.*m_pend.*cos(THE_Theta_pend).*sin(THE_Psi).*sin(THE_Phi_pend).*(2.0./3.0)-(Lx_pend.^2.*THE_Theta_pend_D.*m_pend.*cos(THE_Phi_pend).*cos(THE_Theta_pend).^2.*sin(THE_Psi))./6.0+(Ly_pend.^2.*THE_Psi_pend_D.*m_pend.*cos(THE_Psi).*cos(THE_Phi_pend).^2.*sin(THE_Theta_pend))./6.0+(Ly_pend.^2.*THE_Theta_pend_D.*m_pend.*cos(THE_Phi_pend).*cos(THE_Psi_pend).^2.*sin(THE_Psi))./6.0+(Ly_pend.^2.*THE_Psi_pend_D.*m_pend.*cos(THE_Psi).*cos(THE_Psi_pend).^2.*sin(THE_Theta_pend))./6.0+(Ly_pend.^2.*THE_Theta_pend_D.*m_pend.*cos(THE_Phi_pend).*cos(THE_Theta_pend).^2.*sin(THE_Psi))./6.0-Lz_pend.^2.*THE_Psi_pend_D.*m_pend.*cos(THE_Psi).*cos(THE_Phi_pend).^2.*sin(THE_Theta_pend).*(2.0./3.0)-Lz_pend.^2.*THE_Theta_pend_D.*m_pend.*cos(THE_Phi_pend).*cos(THE_Psi_pend).^2.*sin(THE_Psi).*(2.0./3.0)-Lz_pend.^2.*THE_Psi_pend_D.*m_pend.*cos(THE_Psi).*cos(THE_Psi_pend).^2.*sin(THE_Theta_pend).*(2.0./3.0)-(Lx_pend.^2.*THE_Phi_pend_D.*m_pend.*cos(THE_Psi).*cos(THE_Phi_pend).^2.*cos(THE_Theta_pend).^2)./6.0+(Ly_pend.^2.*THE_Phi_pend_D.*m_pend.*cos(THE_Psi).*cos(THE_Phi_pend).^2.*cos(THE_Psi_pend).^2)./3.0+(Ly_pend.^2.*THE_Phi_pend_D.*m_pend.*cos(THE_Psi).*cos(THE_Phi_pend).^2.*cos(THE_Theta_pend).^2)./6.0-Lz_pend.^2.*THE_Phi_pend_D.*m_pend.*cos(THE_Psi).*cos(THE_Phi_pend).^2.*cos(THE_Psi_pend).^2.*(4.0./3.0)+(Lz_pend.*THE_Psi_D.*Tv_Z_pend.*m_pend.*cos(THE_Psi).*sin(THE_Phi_pend).*sin(THE_Psi_pend))./2.0+(Lx_pend.^2.*THE_Psi_D.*m_pend.*cos(THE_Phi_pend).*cos(THE_Theta_pend).^2.*sin(THE_Psi).*sin(THE_Phi_pend))./1.2e+1-(Ly_pend.^2.*THE_Psi_D.*m_pend.*cos(THE_Phi_pend).*cos(THE_Psi_pend).^2.*sin(THE_Psi).*sin(THE_Phi_pend))./6.0-(Ly_pend.^2.*THE_Psi_D.*m_pend.*cos(THE_Phi_pend).*cos(THE_Theta_pend).^2.*sin(THE_Psi).*sin(THE_Phi_pend))./1.2e+1-(Ly_pend.^2.*THE_Psi_pend_D.*m_pend.*cos(THE_Psi_pend).^2.*cos(THE_Theta_pend).*sin(THE_Psi).*sin(THE_Phi_pend))./6.0+Lz_pend.^2.*THE_Psi_D.*m_pend.*cos(THE_Phi_pend).*cos(THE_Psi_pend).^2.*sin(THE_Psi).*sin(THE_Phi_pend).*(2.0./3.0)+Lz_pend.^2.*THE_Psi_pend_D.*m_pend.*cos(THE_Psi_pend).^2.*cos(THE_Theta_pend).*sin(THE_Psi).*sin(THE_Phi_pend).*(2.0./3.0)-(Ly_pend.^2.*THE_Psi_pend_D.*m_pend.*cos(THE_Psi).*cos(THE_Phi_pend).^2.*cos(THE_Psi_pend).^2.*sin(THE_Theta_pend))./3.0-(Ly_pend.^2.*THE_Theta_pend_D.*m_pend.*cos(THE_Phi_pend).*cos(THE_Psi_pend).^2.*cos(THE_Theta_pend).^2.*sin(THE_Psi))./6.0+Lz_pend.^2.*THE_Psi_pend_D.*m_pend.*cos(THE_Psi).*cos(THE_Phi_pend).^2.*cos(THE_Psi_pend).^2.*sin(THE_Theta_pend).*(4.0./3.0)+Lz_pend.^2.*THE_Theta_pend_D.*m_pend.*cos(THE_Phi_pend).*cos(THE_Psi_pend).^2.*cos(THE_Theta_pend).^2.*sin(THE_Psi).*(2.0./3.0)-(Lx_pend.^2.*THE_Psi_D.*m_pend.*cos(THE_Psi).*cos(THE_Phi_pend).*cos(THE_Theta_pend).*sin(THE_Theta_pend))./1.2e+1+(Ly_pend.^2.*THE_Psi_D.*m_pend.*cos(THE_Psi).*cos(THE_Phi_pend).*cos(THE_Theta_pend).*sin(THE_Theta_pend))./1.2e+1+(Ly_pend.^2.*THE_Theta_pend_D.*m_pend.*cos(THE_Psi).*cos(THE_Psi_pend).*cos(THE_Theta_pend).*sin(THE_Psi_pend))./6.0-Lz_pend.^2.*THE_Theta_pend_D.*m_pend.*cos(THE_Psi).*cos(THE_Psi_pend).*cos(THE_Theta_pend).*sin(THE_Psi_pend).*(2.0./3.0)-(Ly_pend.^2.*THE_Phi_pend_D.*m_pend.*cos(THE_Psi).*cos(THE_Phi_pend).^2.*cos(THE_Psi_pend).^2.*cos(THE_Theta_pend).^2)./6.0+Lz_pend.^2.*THE_Phi_pend_D.*m_pend.*cos(THE_Psi).*cos(THE_Phi_pend).^2.*cos(THE_Psi_pend).^2.*cos(THE_Theta_pend).^2.*(2.0./3.0)-(Ly_pend.^2.*THE_Psi_D.*m_pend.*cos(THE_Psi_pend).*sin(THE_Psi).*sin(THE_Psi_pend).*sin(THE_Theta_pend))./1.2e+1+(Lz_pend.^2.*THE_Psi_D.*m_pend.*cos(THE_Psi_pend).*sin(THE_Psi).*sin(THE_Psi_pend).*sin(THE_Theta_pend))./3.0+(Ly_pend.^2.*THE_Psi_D.*m_pend.*cos(THE_Phi_pend).*cos(THE_Psi_pend).^2.*cos(THE_Theta_pend).^2.*sin(THE_Psi).*sin(THE_Phi_pend))./1.2e+1-(Lz_pend.^2.*THE_Psi_D.*m_pend.*cos(THE_Phi_pend).*cos(THE_Psi_pend).^2.*cos(THE_Theta_pend).^2.*sin(THE_Psi).*sin(THE_Phi_pend))./3.0+(Lx_pend.^2.*THE_Theta_pend_D.*m_pend.*cos(THE_Psi).*cos(THE_Phi_pend).*cos(THE_Theta_pend).*sin(THE_Phi_pend).*sin(THE_Theta_pend))./6.0-(Ly_pend.^2.*THE_Psi_D.*m_pend.*cos(THE_Psi).*cos(THE_Psi_pend).*cos(THE_Theta_pend).*sin(THE_Phi_pend).*sin(THE_Psi_pend))./1.2e+1-(Ly_pend.^2.*THE_Psi_pend_D.*m_pend.*cos(THE_Psi).*cos(THE_Phi_pend).*cos(THE_Psi_pend).*sin(THE_Phi_pend).*sin(THE_Psi_pend))./3.0-(Ly_pend.^2.*THE_Theta_pend_D.*m_pend.*cos(THE_Psi).*cos(THE_Phi_pend).*cos(THE_Theta_pend).*sin(THE_Phi_pend).*sin(THE_Theta_pend))./6.0+(Lz_pend.^2.*THE_Psi_D.*m_pend.*cos(THE_Psi).*cos(THE_Psi_pend).*cos(THE_Theta_pend).*sin(THE_Phi_pend).*sin(THE_Psi_pend))./3.0+Lz_pend.^2.*THE_Psi_pend_D.*m_pend.*cos(THE_Psi).*cos(THE_Phi_pend).*cos(THE_Psi_pend).*sin(THE_Phi_pend).*sin(THE_Psi_pend).*(4.0./3.0)+(Ly_pend.^2.*THE_Theta_pend_D.*m_pend.*cos(THE_Psi_pend).*sin(THE_Psi).*sin(THE_Phi_pend).*sin(THE_Psi_pend).*sin(THE_Theta_pend))./6.0-Lz_pend.^2.*THE_Theta_pend_D.*m_pend.*cos(THE_Psi_pend).*sin(THE_Psi).*sin(THE_Phi_pend).*sin(THE_Psi_pend).*sin(THE_Theta_pend).*(2.0./3.0)+(Lz_pend.*THE_Psi_D.*Tv_Z_pend.*m_pend.*cos(THE_Psi).*cos(THE_Phi_pend).*cos(THE_Psi_pend).*sin(THE_Theta_pend))./2.0-(Ly_pend.^2.*THE_Psi_D.*m_pend.*cos(THE_Psi).*cos(THE_Phi_pend).*cos(THE_Psi_pend).^2.*cos(THE_Theta_pend).*sin(THE_Theta_pend))./1.2e+1-(Ly_pend.^2.*THE_Theta_pend_D.*m_pend.*cos(THE_Psi).*cos(THE_Phi_pend).^2.*cos(THE_Psi_pend).*cos(THE_Theta_pend).*sin(THE_Psi_pend))./6.0+(Lz_pend.^2.*THE_Psi_D.*m_pend.*cos(THE_Psi).*cos(THE_Phi_pend).*cos(THE_Psi_pend).^2.*cos(THE_Theta_pend).*sin(THE_Theta_pend))./3.0+Lz_pend.^2.*THE_Theta_pend_D.*m_pend.*cos(THE_Psi).*cos(THE_Phi_pend).^2.*cos(THE_Psi_pend).*cos(THE_Theta_pend).*sin(THE_Psi_pend).*(2.0./3.0)+(Ly_pend.^2.*THE_Psi_D.*m_pend.*cos(THE_Phi_pend).^2.*cos(THE_Psi_pend).*sin(THE_Psi).*sin(THE_Psi_pend).*sin(THE_Theta_pend))./6.0-Lz_pend.^2.*THE_Psi_D.*m_pend.*cos(THE_Phi_pend).^2.*cos(THE_Psi_pend).*sin(THE_Psi).*sin(THE_Psi_pend).*sin(THE_Theta_pend).*(2.0./3.0)+(Ly_pend.^2.*THE_Phi_pend_D.*m_pend.*cos(THE_Psi).*cos(THE_Phi_pend).*cos(THE_Psi_pend).*sin(THE_Phi_pend).*sin(THE_Psi_pend).*sin(THE_Theta_pend))./3.0+(Ly_pend.^2.*THE_Psi_pend_D.*m_pend.*cos(THE_Phi_pend).*cos(THE_Psi_pend).*cos(THE_Theta_pend).*sin(THE_Psi).*sin(THE_Psi_pend).*sin(THE_Theta_pend))./6.0-Lz_pend.^2.*THE_Phi_pend_D.*m_pend.*cos(THE_Psi).*cos(THE_Phi_pend).*cos(THE_Psi_pend).*sin(THE_Phi_pend).*sin(THE_Psi_pend).*sin(THE_Theta_pend).*(4.0./3.0)-Lz_pend.^2.*THE_Psi_pend_D.*m_pend.*cos(THE_Phi_pend).*cos(THE_Psi_pend).*cos(THE_Theta_pend).*sin(THE_Psi).*sin(THE_Psi_pend).*sin(THE_Theta_pend).*(2.0./3.0)+(Ly_pend.^2.*THE_Psi_pend_D.*m_pend.*cos(THE_Psi).*cos(THE_Phi_pend).*cos(THE_Psi_pend).*cos(THE_Theta_pend).^2.*sin(THE_Phi_pend).*sin(THE_Psi_pend))./6.0+(Ly_pend.^2.*THE_Theta_pend_D.*m_pend.*cos(THE_Psi).*cos(THE_Phi_pend).*cos(THE_Psi_pend).^2.*cos(THE_Theta_pend).*sin(THE_Phi_pend).*sin(THE_Theta_pend))./6.0-Lz_pend.^2.*THE_Psi_pend_D.*m_pend.*cos(THE_Psi).*cos(THE_Phi_pend).*cos(THE_Psi_pend).*cos(THE_Theta_pend).^2.*sin(THE_Phi_pend).*sin(THE_Psi_pend).*(2.0./3.0)-Lz_pend.^2.*THE_Theta_pend_D.*m_pend.*cos(THE_Psi).*cos(THE_Phi_pend).*cos(THE_Psi_pend).^2.*cos(THE_Theta_pend).*sin(THE_Phi_pend).*sin(THE_Theta_pend).*(2.0./3.0),(Ly_pend.^2.*THE_Phi_pend_D.*m_pend.*sin(THE_Phi_pend.*2.0))./1.2e+1+(Ly_pend.^2.*THE_Psi_pend_D.*m_pend.*sin(THE_Psi_pend.*2.0))./1.2e+1-(Lz_pend.^2.*THE_Phi_pend_D.*m_pend.*sin(THE_Phi_pend.*2.0))./3.0-(Lz_pend.^2.*THE_Psi_pend_D.*m_pend.*sin(THE_Psi_pend.*2.0))./3.0-(Ly_pend.^2.*THE_Psi_pend_D.*m_pend.*cos(THE_Phi_pend).*sin(THE_Phi_pend).*sin(THE_Theta_pend))./6.0-(Ly_pend.^2.*THE_Phi_pend_D.*m_pend.*cos(THE_Psi_pend).*sin(THE_Psi_pend).*sin(THE_Theta_pend))./6.0+Lz_pend.^2.*THE_Psi_pend_D.*m_pend.*cos(THE_Phi_pend).*sin(THE_Phi_pend).*sin(THE_Theta_pend).*(2.0./3.0)+Lz_pend.^2.*THE_Phi_pend_D.*m_pend.*cos(THE_Psi_pend).*sin(THE_Psi_pend).*sin(THE_Theta_pend).*(2.0./3.0)-Lz_pend.*THE_Psi_pend_D.*Tv_Z_pend.*m_pend.*cos(THE_Theta_pend).*sin(THE_Psi_pend)-Lz_pend.*THE_Theta_pend_D.*Tv_Z_pend.*m_pend.*cos(THE_Psi_pend).*sin(THE_Theta_pend)+(Lx_pend.^2.*THE_Phi_pend_D.*m_pend.*cos(THE_Phi_pend).*cos(THE_Theta_pend).^2.*sin(THE_Phi_pend))./6.0+(Lx_pend.^2.*THE_Theta_pend_D.*m_pend.*cos(THE_Phi_pend).^2.*cos(THE_Theta_pend).*sin(THE_Theta_pend))./6.0-(Ly_pend.^2.*THE_Phi_pend_D.*m_pend.*cos(THE_Phi_pend).*cos(THE_Psi_pend).^2.*sin(THE_Phi_pend))./3.0-(Ly_pend.^2.*THE_Psi_pend_D.*m_pend.*cos(THE_Phi_pend).^2.*cos(THE_Psi_pend).*sin(THE_Psi_pend))./3.0-(Ly_pend.^2.*THE_Phi_pend_D.*m_pend.*cos(THE_Phi_pend).*cos(THE_Theta_pend).^2.*sin(THE_Phi_pend))./6.0-(Ly_pend.^2.*THE_Theta_pend_D.*m_pend.*cos(THE_Phi_pend).^2.*cos(THE_Theta_pend).*sin(THE_Theta_pend))./6.0+Lz_pend.^2.*THE_Phi_pend_D.*m_pend.*cos(THE_Phi_pend).*cos(THE_Psi_pend).^2.*sin(THE_Phi_pend).*(4.0./3.0)+Lz_pend.^2.*THE_Psi_pend_D.*m_pend.*cos(THE_Phi_pend).^2.*cos(THE_Psi_pend).*sin(THE_Psi_pend).*(4.0./3.0)+(Ly_pend.^2.*THE_Phi_pend_D.*m_pend.*cos(THE_Phi_pend).^2.*cos(THE_Psi_pend).*sin(THE_Psi_pend).*sin(THE_Theta_pend))./3.0+(Ly_pend.^2.*THE_Psi_pend_D.*m_pend.*cos(THE_Phi_pend).*cos(THE_Psi_pend).^2.*sin(THE_Phi_pend).*sin(THE_Theta_pend))./3.0-Lz_pend.^2.*THE_Phi_pend_D.*m_pend.*cos(THE_Phi_pend).^2.*cos(THE_Psi_pend).*sin(THE_Psi_pend).*sin(THE_Theta_pend).*(4.0./3.0)-Lz_pend.^2.*THE_Psi_pend_D.*m_pend.*cos(THE_Phi_pend).*cos(THE_Psi_pend).^2.*sin(THE_Phi_pend).*sin(THE_Theta_pend).*(4.0./3.0)+(Ly_pend.^2.*THE_Phi_pend_D.*m_pend.*cos(THE_Phi_pend).*cos(THE_Psi_pend).^2.*cos(THE_Theta_pend).^2.*sin(THE_Phi_pend))./6.0+(Ly_pend.^2.*THE_Psi_pend_D.*m_pend.*cos(THE_Phi_pend).^2.*cos(THE_Psi_pend).*cos(THE_Theta_pend).^2.*sin(THE_Psi_pend))./6.0+(Ly_pend.^2.*THE_Theta_pend_D.*m_pend.*cos(THE_Phi_pend).^2.*cos(THE_Psi_pend).^2.*cos(THE_Theta_pend).*sin(THE_Theta_pend))./6.0-Lz_pend.^2.*THE_Phi_pend_D.*m_pend.*cos(THE_Phi_pend).*cos(THE_Psi_pend).^2.*cos(THE_Theta_pend).^2.*sin(THE_Phi_pend).*(2.0./3.0)-Lz_pend.^2.*THE_Psi_pend_D.*m_pend.*cos(THE_Phi_pend).^2.*cos(THE_Psi_pend).*cos(THE_Theta_pend).^2.*sin(THE_Psi_pend).*(2.0./3.0)-Lz_pend.^2.*THE_Theta_pend_D.*m_pend.*cos(THE_Phi_pend).^2.*cos(THE_Psi_pend).^2.*cos(THE_Theta_pend).*sin(THE_Theta_pend).*(2.0./3.0)+(Ly_pend.^2.*THE_Theta_pend_D.*m_pend.*cos(THE_Phi_pend).*cos(THE_Psi_pend).*cos(THE_Theta_pend).*sin(THE_Phi_pend).*sin(THE_Psi_pend))./6.0-Lz_pend.^2.*THE_Theta_pend_D.*m_pend.*cos(THE_Phi_pend).*cos(THE_Psi_pend).*cos(THE_Theta_pend).*sin(THE_Phi_pend).*sin(THE_Psi_pend).*(2.0./3.0),-THE_Psi_D.*Tv_Z_pend.*m_pend.*sin(THE_Phi).*sin(THE_Psi)-THE_Psi_D.*cg_to_mot_H.*mprop.*sin(THE_Phi).*sin(THE_Psi).*4.0-THE_Psi_D.*Tv_Z_pend.*m_pend.*cos(THE_Phi).*cos(THE_Psi).*sin(THE_Theta)-THE_Psi_D.*cg_to_mot_H.*mprop.*cos(THE_Phi).*cos(THE_Psi).*sin(THE_Theta).*4.0-(Lz_pend.*THE_Psi_D.*m_pend.*cos(THE_Psi).*cos(THE_Phi_pend).*sin(THE_Phi).*sin(THE_Psi_pend))./2.0-(Lz_pend.*THE_Psi_D.*m_pend.*cos(THE_Psi_pend).*cos(THE_Theta_pend).*sin(THE_Phi).*sin(THE_Psi))./2.0-Lz_pend.*THE_Psi_pend_D.*m_pend.*cos(THE_Phi_pend).*cos(THE_Psi_pend).*sin(THE_Phi).*sin(THE_Psi)-Lz_pend.*THE_Psi_pend_D.*m_pend.*cos(THE_Psi).*cos(THE_Theta_pend).*sin(THE_Phi).*sin(THE_Psi_pend)-Lz_pend.*THE_Theta_pend_D.*m_pend.*cos(THE_Psi).*cos(THE_Psi_pend).*sin(THE_Phi).*sin(THE_Theta_pend)+Lz_pend.*THE_Phi_pend_D.*m_pend.*sin(THE_Phi).*sin(THE_Psi).*sin(THE_Phi_pend).*sin(THE_Psi_pend)-(Lz_pend.*THE_Psi_D.*m_pend.*cos(THE_Phi).*cos(THE_Psi).*cos(THE_Psi_pend).*cos(THE_Theta_pend).*sin(THE_Theta))./2.0-Lz_pend.*THE_Psi_pend_D.*m_pend.*cos(THE_Phi).*cos(THE_Psi).*cos(THE_Phi_pend).*cos(THE_Psi_pend).*sin(THE_Theta)+(Lz_pend.*THE_Psi_D.*m_pend.*cos(THE_Phi).*cos(THE_Phi_pend).*sin(THE_Psi).*sin(THE_Theta).*sin(THE_Psi_pend))./2.0+Lz_pend.*THE_Phi_pend_D.*m_pend.*cos(THE_Phi).*cos(THE_Psi).*sin(THE_Theta).*sin(THE_Phi_pend).*sin(THE_Psi_pend)+(Lz_pend.*THE_Psi_D.*m_pend.*cos(THE_Psi).*cos(THE_Psi_pend).*sin(THE_Phi).*sin(THE_Phi_pend).*sin(THE_Theta_pend))./2.0+Lz_pend.*THE_Psi_pend_D.*m_pend.*cos(THE_Phi).*cos(THE_Theta_pend).*sin(THE_Psi).*sin(THE_Theta).*sin(THE_Psi_pend)+Lz_pend.*THE_Theta_pend_D.*m_pend.*cos(THE_Phi).*cos(THE_Psi_pend).*sin(THE_Psi).*sin(THE_Theta).*sin(THE_Theta_pend)+Lz_pend.*THE_Phi_pend_D.*m_pend.*cos(THE_Phi_pend).*cos(THE_Psi_pend).*sin(THE_Phi).*sin(THE_Psi).*sin(THE_Theta_pend)+Lz_pend.*THE_Theta_pend_D.*m_pend.*cos(THE_Psi_pend).*cos(THE_Theta_pend).*sin(THE_Phi).*sin(THE_Psi).*sin(THE_Phi_pend)-Lz_pend.*THE_Psi_pend_D.*m_pend.*sin(THE_Phi).*sin(THE_Psi).*sin(THE_Phi_pend).*sin(THE_Psi_pend).*sin(THE_Theta_pend)+Lz_pend.*THE_Phi_pend_D.*m_pend.*cos(THE_Phi).*cos(THE_Psi).*cos(THE_Phi_pend).*cos(THE_Psi_pend).*sin(THE_Theta).*sin(THE_Theta_pend)+Lz_pend.*THE_Theta_pend_D.*m_pend.*cos(THE_Phi).*cos(THE_Psi).*cos(THE_Psi_pend).*cos(THE_Theta_pend).*sin(THE_Theta).*sin(THE_Phi_pend)-(Lz_pend.*THE_Psi_D.*m_pend.*cos(THE_Phi).*cos(THE_Psi_pend).*sin(THE_Psi).*sin(THE_Theta).*sin(THE_Phi_pend).*sin(THE_Theta_pend))./2.0-Lz_pend.*THE_Psi_pend_D.*m_pend.*cos(THE_Phi).*cos(THE_Psi).*sin(THE_Theta).*sin(THE_Phi_pend).*sin(THE_Psi_pend).*sin(THE_Theta_pend),THE_Psi_D.*cg_to_mot_H.*mprop.*cos(THE_Phi).*sin(THE_Psi).*4.0+THE_Psi_D.*Tv_Z_pend.*m_pend.*cos(THE_Phi).*sin(THE_Psi)-THE_Psi_D.*Tv_Z_pend.*m_pend.*cos(THE_Psi).*sin(THE_Phi).*sin(THE_Theta)-THE_Psi_D.*cg_to_mot_H.*mprop.*cos(THE_Psi).*sin(THE_Phi).*sin(THE_Theta).*4.0+(Lz_pend.*THE_Psi_D.*m_pend.*cos(THE_Phi).*cos(THE_Psi).*cos(THE_Phi_pend).*sin(THE_Psi_pend))./2.0+(Lz_pend.*THE_Psi_D.*m_pend.*cos(THE_Phi).*cos(THE_Psi_pend).*cos(THE_Theta_pend).*sin(THE_Psi))./2.0+Lz_pend.*THE_Psi_pend_D.*m_pend.*cos(THE_Phi).*cos(THE_Phi_pend).*cos(THE_Psi_pend).*sin(THE_Psi)+Lz_pend.*THE_Psi_pend_D.*m_pend.*cos(THE_Phi).*cos(THE_Psi).*cos(THE_Theta_pend).*sin(THE_Psi_pend)+Lz_pend.*THE_Theta_pend_D.*m_pend.*cos(THE_Phi).*cos(THE_Psi).*cos(THE_Psi_pend).*sin(THE_Theta_pend)-Lz_pend.*THE_Phi_pend_D.*m_pend.*cos(THE_Phi).*sin(THE_Psi).*sin(THE_Phi_pend).*sin(THE_Psi_pend)-(Lz_pend.*THE_Psi_D.*m_pend.*cos(THE_Psi).*cos(THE_Psi_pend).*cos(THE_Theta_pend).*sin(THE_Phi).*sin(THE_Theta))./2.0-(Lz_pend.*THE_Psi_D.*m_pend.*cos(THE_Phi).*cos(THE_Psi).*cos(THE_Psi_pend).*sin(THE_Phi_pend).*sin(THE_Theta_pend))./2.0-Lz_pend.*THE_Psi_pend_D.*m_pend.*cos(THE_Psi).*cos(THE_Phi_pend).*cos(THE_Psi_pend).*sin(THE_Phi).*sin(THE_Theta)-Lz_pend.*THE_Phi_pend_D.*m_pend.*cos(THE_Phi).*cos(THE_Phi_pend).*cos(THE_Psi_pend).*sin(THE_Psi).*sin(THE_Theta_pend)-Lz_pend.*THE_Theta_pend_D.*m_pend.*cos(THE_Phi).*cos(THE_Psi_pend).*cos(THE_Theta_pend).*sin(THE_Psi).*sin(THE_Phi_pend)+(Lz_pend.*THE_Psi_D.*m_pend.*cos(THE_Phi_pend).*sin(THE_Phi).*sin(THE_Psi).*sin(THE_Theta).*sin(THE_Psi_pend))./2.0+Lz_pend.*THE_Phi_pend_D.*m_pend.*cos(THE_Psi).*sin(THE_Phi).*sin(THE_Theta).*sin(THE_Phi_pend).*sin(THE_Psi_pend)+Lz_pend.*THE_Psi_pend_D.*m_pend.*cos(THE_Theta_pend).*sin(THE_Phi).*sin(THE_Psi).*sin(THE_Theta).*sin(THE_Psi_pend)+Lz_pend.*THE_Theta_pend_D.*m_pend.*cos(THE_Psi_pend).*sin(THE_Phi).*sin(THE_Psi).*sin(THE_Theta).*sin(THE_Theta_pend)+Lz_pend.*THE_Psi_pend_D.*m_pend.*cos(THE_Phi).*sin(THE_Psi).*sin(THE_Phi_pend).*sin(THE_Psi_pend).*sin(THE_Theta_pend)-(Lz_pend.*THE_Psi_D.*m_pend.*cos(THE_Psi_pend).*sin(THE_Phi).*sin(THE_Psi).*sin(THE_Theta).*sin(THE_Phi_pend).*sin(THE_Theta_pend))./2.0-Lz_pend.*THE_Psi_pend_D.*m_pend.*cos(THE_Psi).*sin(THE_Phi).*sin(THE_Theta).*sin(THE_Phi_pend).*sin(THE_Psi_pend).*sin(THE_Theta_pend)+Lz_pend.*THE_Phi_pend_D.*m_pend.*cos(THE_Psi).*cos(THE_Phi_pend).*cos(THE_Psi_pend).*sin(THE_Phi).*sin(THE_Theta).*sin(THE_Theta_pend)+Lz_pend.*THE_Theta_pend_D.*m_pend.*cos(THE_Psi).*cos(THE_Psi_pend).*cos(THE_Theta_pend).*sin(THE_Phi).*sin(THE_Theta).*sin(THE_Phi_pend),cos(THE_Theta).*(THE_Psi_D.*Tv_Z_pend.*m_pend.*cos(THE_Psi).*2.0+THE_Psi_D.*cg_to_mot_H.*mprop.*cos(THE_Psi).*8.0+Lz_pend.*THE_Psi_D.*m_pend.*cos(THE_Psi).*cos(THE_Psi_pend).*cos(THE_Theta_pend)+Lz_pend.*THE_Psi_pend_D.*m_pend.*cos(THE_Psi).*cos(THE_Phi_pend).*cos(THE_Psi_pend).*2.0-Lz_pend.*THE_Psi_D.*m_pend.*cos(THE_Phi_pend).*sin(THE_Psi).*sin(THE_Psi_pend)-Lz_pend.*THE_Phi_pend_D.*m_pend.*cos(THE_Psi).*sin(THE_Phi_pend).*sin(THE_Psi_pend).*2.0-Lz_pend.*THE_Psi_pend_D.*m_pend.*cos(THE_Theta_pend).*sin(THE_Psi).*sin(THE_Psi_pend).*2.0-Lz_pend.*THE_Theta_pend_D.*m_pend.*cos(THE_Psi_pend).*sin(THE_Psi).*sin(THE_Theta_pend).*2.0-Lz_pend.*THE_Phi_pend_D.*m_pend.*cos(THE_Psi).*cos(THE_Phi_pend).*cos(THE_Psi_pend).*sin(THE_Theta_pend).*2.0-Lz_pend.*THE_Theta_pend_D.*m_pend.*cos(THE_Psi).*cos(THE_Psi_pend).*cos(THE_Theta_pend).*sin(THE_Phi_pend).*2.0+Lz_pend.*THE_Psi_D.*m_pend.*cos(THE_Psi_pend).*sin(THE_Psi).*sin(THE_Phi_pend).*sin(THE_Theta_pend)+Lz_pend.*THE_Psi_pend_D.*m_pend.*cos(THE_Psi).*sin(THE_Phi_pend).*sin(THE_Psi_pend).*sin(THE_Theta_pend).*2.0).*(-1.0./2.0),(m_pend.*(Ly_pend.^2.*THE_Theta_pend_D.*cos(THE_Phi_pend).*2.0-(Ly_pend.^2.*THE_Psi_D.*sin(THE_Phi_pend.*2.0))./2.0+Lz_pend.^2.*THE_Psi_D.*sin(THE_Phi_pend.*2.0).*2.0+Lx_pend.^2.*THE_Theta_pend_D.*cos(THE_Phi_pend).*cos(THE_Theta_pend).^2.*2.0-Ly_pend.^2.*THE_Theta_pend_D.*cos(THE_Phi_pend).*cos(THE_Psi_pend).^2.*2.0-Ly_pend.^2.*THE_Theta_pend_D.*cos(THE_Phi_pend).*cos(THE_Theta_pend).^2.*2.0+Lz_pend.^2.*THE_Theta_pend_D.*cos(THE_Phi_pend).*cos(THE_Psi_pend).^2.*8.0+Lz_pend.^2.*THE_Psi_pend_D.*cos(THE_Theta_pend).*sin(THE_Phi_pend).*8.0+Ly_pend.^2.*THE_Theta_pend_D.*cos(THE_Phi_pend).*cos(THE_Psi_pend).^2.*cos(THE_Theta_pend).^2.*2.0-Lz_pend.^2.*THE_Theta_pend_D.*cos(THE_Phi_pend).*cos(THE_Psi_pend).^2.*cos(THE_Theta_pend).^2.*8.0+Ly_pend.^2.*THE_Psi_D.*cos(THE_Psi_pend).*sin(THE_Psi_pend).*sin(THE_Theta_pend)-Lz_pend.^2.*THE_Psi_D.*cos(THE_Psi_pend).*sin(THE_Psi_pend).*sin(THE_Theta_pend).*4.0-Lx_pend.^2.*THE_Psi_D.*cos(THE_Phi_pend).*cos(THE_Theta_pend).^2.*sin(THE_Phi_pend)+Ly_pend.^2.*THE_Psi_D.*cos(THE_Phi_pend).*cos(THE_Psi_pend).^2.*sin(THE_Phi_pend).*2.0+Ly_pend.^2.*THE_Psi_D.*cos(THE_Phi_pend).*cos(THE_Theta_pend).^2.*sin(THE_Phi_pend)+Ly_pend.^2.*THE_Psi_pend_D.*cos(THE_Psi_pend).^2.*cos(THE_Theta_pend).*sin(THE_Phi_pend).*2.0-Lz_pend.^2.*THE_Psi_D.*cos(THE_Phi_pend).*cos(THE_Psi_pend).^2.*sin(THE_Phi_pend).*8.0-Lz_pend.^2.*THE_Psi_pend_D.*cos(THE_Psi_pend).^2.*cos(THE_Theta_pend).*sin(THE_Phi_pend).*8.0-Ly_pend.^2.*THE_Psi_D.*cos(THE_Phi_pend).*cos(THE_Psi_pend).^2.*cos(THE_Theta_pend).^2.*sin(THE_Phi_pend)+Lz_pend.^2.*THE_Psi_D.*cos(THE_Phi_pend).*cos(THE_Psi_pend).^2.*cos(THE_Theta_pend).^2.*sin(THE_Phi_pend).*4.0-Ly_pend.^2.*THE_Theta_pend_D.*cos(THE_Psi_pend).*sin(THE_Phi_pend).*sin(THE_Psi_pend).*sin(THE_Theta_pend).*2.0+Lz_pend.^2.*THE_Theta_pend_D.*cos(THE_Psi_pend).*sin(THE_Phi_pend).*sin(THE_Psi_pend).*sin(THE_Theta_pend).*8.0-Ly_pend.^2.*THE_Psi_D.*cos(THE_Phi_pend).^2.*cos(THE_Psi_pend).*sin(THE_Psi_pend).*sin(THE_Theta_pend).*2.0+Lz_pend.^2.*THE_Psi_D.*cos(THE_Phi_pend).^2.*cos(THE_Psi_pend).*sin(THE_Psi_pend).*sin(THE_Theta_pend).*8.0-Ly_pend.^2.*THE_Psi_pend_D.*cos(THE_Phi_pend).*cos(THE_Psi_pend).*cos(THE_Theta_pend).*sin(THE_Psi_pend).*sin(THE_Theta_pend).*2.0+Lz_pend.^2.*THE_Psi_pend_D.*cos(THE_Phi_pend).*cos(THE_Psi_pend).*cos(THE_Theta_pend).*sin(THE_Psi_pend).*sin(THE_Theta_pend).*8.0))./1.2e+1,Ly_pend.^2.*THE_Phi_pend_D.*m_pend.*cos(THE_Phi_pend).*(-1.0./6.0)+(Ly_pend.^2.*THE_Psi_pend_D.*m_pend.*cos(THE_Phi_pend).*sin(THE_Theta_pend))./6.0-(Lx_pend.^2.*THE_Phi_pend_D.*m_pend.*cos(THE_Phi_pend).*cos(THE_Theta_pend).^2)./6.0+(Ly_pend.^2.*THE_Phi_pend_D.*m_pend.*cos(THE_Phi_pend).*cos(THE_Psi_pend).^2)./6.0+(Ly_pend.^2.*THE_Phi_pend_D.*m_pend.*cos(THE_Phi_pend).*cos(THE_Theta_pend).^2)./6.0-Lz_pend.^2.*THE_Phi_pend_D.*m_pend.*cos(THE_Phi_pend).*cos(THE_Psi_pend).^2.*(2.0./3.0)-(Ly_pend.^2.*THE_Psi_pend_D.*m_pend.*cos(THE_Psi_pend).*sin(THE_Phi_pend).*sin(THE_Psi_pend))./6.0+Lz_pend.^2.*THE_Psi_pend_D.*m_pend.*cos(THE_Psi_pend).*sin(THE_Phi_pend).*sin(THE_Psi_pend).*(2.0./3.0)+(Lz_pend.*THE_Psi_D.*Tv_Z_pend.*m_pend.*cos(THE_Psi_pend).*sin(THE_Theta_pend))./2.0-(Lx_pend.^2.*THE_Psi_D.*m_pend.*cos(THE_Phi_pend).^2.*cos(THE_Theta_pend).*sin(THE_Theta_pend))./1.2e+1+(Ly_pend.^2.*THE_Psi_D.*m_pend.*cos(THE_Phi_pend).^2.*cos(THE_Theta_pend).*sin(THE_Theta_pend))./1.2e+1-(Ly_pend.^2.*THE_Psi_pend_D.*m_pend.*cos(THE_Phi_pend).*cos(THE_Psi_pend).^2.*sin(THE_Theta_pend))./6.0+Lz_pend.^2.*THE_Psi_pend_D.*m_pend.*cos(THE_Phi_pend).*cos(THE_Psi_pend).^2.*sin(THE_Theta_pend).*(2.0./3.0)-(Ly_pend.^2.*THE_Phi_pend_D.*m_pend.*cos(THE_Phi_pend).*cos(THE_Psi_pend).^2.*cos(THE_Theta_pend).^2)./6.0+Lz_pend.^2.*THE_Phi_pend_D.*m_pend.*cos(THE_Phi_pend).*cos(THE_Psi_pend).^2.*cos(THE_Theta_pend).^2.*(2.0./3.0)-(Ly_pend.^2.*THE_Psi_D.*m_pend.*cos(THE_Phi_pend).^2.*cos(THE_Psi_pend).^2.*cos(THE_Theta_pend).*sin(THE_Theta_pend))./1.2e+1+(Lz_pend.^2.*THE_Psi_D.*m_pend.*cos(THE_Phi_pend).^2.*cos(THE_Psi_pend).^2.*cos(THE_Theta_pend).*sin(THE_Theta_pend))./3.0+(Ly_pend.^2.*THE_Phi_pend_D.*m_pend.*cos(THE_Psi_pend).*sin(THE_Phi_pend).*sin(THE_Psi_pend).*sin(THE_Theta_pend))./6.0-Lz_pend.^2.*THE_Phi_pend_D.*m_pend.*cos(THE_Psi_pend).*sin(THE_Phi_pend).*sin(THE_Psi_pend).*sin(THE_Theta_pend).*(2.0./3.0)-(Ly_pend.^2.*THE_Psi_D.*m_pend.*cos(THE_Phi_pend).*cos(THE_Psi_pend).*cos(THE_Theta_pend).*sin(THE_Phi_pend).*sin(THE_Psi_pend))./1.2e+1+(Lz_pend.^2.*THE_Psi_D.*m_pend.*cos(THE_Phi_pend).*cos(THE_Psi_pend).*cos(THE_Theta_pend).*sin(THE_Phi_pend).*sin(THE_Psi_pend))./3.0,m_pend.*((Ly_pend.^2.*THE_Psi_D.*sin(THE_Psi_pend.*2.0))./2.0-Lz_pend.^2.*THE_Psi_D.*sin(THE_Psi_pend.*2.0).*2.0+Ly_pend.^2.*THE_Theta_pend_D.*cos(THE_Phi_pend).*sin(THE_Theta_pend).*2.0+Lz_pend.^2.*THE_Phi_pend_D.*cos(THE_Theta_pend).*sin(THE_Phi_pend).*8.0-Ly_pend.^2.*THE_Psi_D.*cos(THE_Phi_pend).*sin(THE_Phi_pend).*sin(THE_Theta_pend)-Ly_pend.^2.*THE_Theta_pend_D.*cos(THE_Psi_pend).*sin(THE_Phi_pend).*sin(THE_Psi_pend).*2.0+Lz_pend.^2.*THE_Psi_D.*cos(THE_Phi_pend).*sin(THE_Phi_pend).*sin(THE_Theta_pend).*4.0+Lz_pend.^2.*THE_Theta_pend_D.*cos(THE_Psi_pend).*sin(THE_Phi_pend).*sin(THE_Psi_pend).*8.0-Lz_pend.*THE_Psi_D.*Tv_Z_pend.*cos(THE_Theta_pend).*sin(THE_Psi_pend).*6.0-Ly_pend.^2.*THE_Psi_D.*cos(THE_Phi_pend).^2.*cos(THE_Psi_pend).*sin(THE_Psi_pend).*2.0+Ly_pend.^2.*THE_Phi_pend_D.*cos(THE_Psi_pend).^2.*cos(THE_Theta_pend).*sin(THE_Phi_pend).*2.0-Ly_pend.^2.*THE_Theta_pend_D.*cos(THE_Phi_pend).*cos(THE_Psi_pend).^2.*sin(THE_Theta_pend).*2.0+Lz_pend.^2.*THE_Psi_D.*cos(THE_Phi_pend).^2.*cos(THE_Psi_pend).*sin(THE_Psi_pend).*8.0-Lz_pend.^2.*THE_Phi_pend_D.*cos(THE_Psi_pend).^2.*cos(THE_Theta_pend).*sin(THE_Phi_pend).*8.0+Lz_pend.^2.*THE_Theta_pend_D.*cos(THE_Phi_pend).*cos(THE_Psi_pend).^2.*sin(THE_Theta_pend).*8.0+Ly_pend.^2.*THE_Psi_D.*cos(THE_Phi_pend).^2.*cos(THE_Psi_pend).*cos(THE_Theta_pend).^2.*sin(THE_Psi_pend)-Lz_pend.^2.*THE_Psi_D.*cos(THE_Phi_pend).^2.*cos(THE_Psi_pend).*cos(THE_Theta_pend).^2.*sin(THE_Psi_pend).*4.0+Ly_pend.^2.*THE_Psi_D.*cos(THE_Phi_pend).*cos(THE_Psi_pend).^2.*sin(THE_Phi_pend).*sin(THE_Theta_pend).*2.0-Lz_pend.^2.*THE_Psi_D.*cos(THE_Phi_pend).*cos(THE_Psi_pend).^2.*sin(THE_Phi_pend).*sin(THE_Theta_pend).*8.0-Ly_pend.^2.*THE_Phi_pend_D.*cos(THE_Phi_pend).*cos(THE_Psi_pend).*cos(THE_Theta_pend).*sin(THE_Psi_pend).*sin(THE_Theta_pend).*2.0+Lz_pend.^2.*THE_Phi_pend_D.*cos(THE_Phi_pend).*cos(THE_Psi_pend).*cos(THE_Theta_pend).*sin(THE_Psi_pend).*sin(THE_Theta_pend).*8.0).*(-1.0./1.2e+1),0.0,0.0,0.0,0.0,0.0,0.0,0.0,0.0,0.0,0.0,0.0,0.0,0.0,0.0,0.0,0.0,0.0,0.0,0.0,0.0,0.0,0.0,0.0,0.0,0.0,0.0,0.0,(Lx_pend.^2.*THE_Theta_pend_D.*m_pend.*cos(THE_Phi_pend).*sin(THE_Theta))./6.0-(Lx_pend.^2.*THE_Theta_pend_D.*m_pend.*cos(THE_Theta).*sin(THE_Psi).*sin(THE_Phi_pend))./6.0+(Ly_pend.^2.*THE_Psi_pend_D.*m_pend.*cos(THE_Theta_pend).*sin(THE_Theta).*sin(THE_Phi_pend))./6.0-(Lx_pend.^2.*THE_Theta_pend_D.*m_pend.*cos(THE_Phi_pend).*cos(THE_Theta_pend).^2.*sin(THE_Theta))./6.0+(Ly_pend.^2.*THE_Theta_pend_D.*m_pend.*cos(THE_Phi_pend).*cos(THE_Theta_pend).^2.*sin(THE_Theta))./6.0+(Lz_pend.*THE_Phi_pend_D.*Tv_Z_pend.*m_pend.*cos(THE_Phi_pend).*sin(THE_Theta).*sin(THE_Psi_pend))./2.0+Lz_pend.*THE_Psi_pend_D.*Tv_Z_pend.*m_pend.*cos(THE_Psi_pend).*sin(THE_Theta).*sin(THE_Phi_pend)+(Lx_pend.^2.*THE_Theta_pend_D.*m_pend.*cos(THE_Theta).*cos(THE_Theta_pend).^2.*sin(THE_Psi).*sin(THE_Phi_pend))./6.0-(Ly_pend.^2.*THE_Theta_pend_D.*m_pend.*cos(THE_Theta).*cos(THE_Theta_pend).^2.*sin(THE_Psi).*sin(THE_Phi_pend))./6.0-(Ly_pend.^2.*THE_Psi_pend_D.*m_pend.*cos(THE_Psi_pend).^2.*cos(THE_Theta_pend).*sin(THE_Theta).*sin(THE_Phi_pend))./6.0+Lz_pend.^2.*THE_Psi_pend_D.*m_pend.*cos(THE_Psi_pend).^2.*cos(THE_Theta_pend).*sin(THE_Theta).*sin(THE_Phi_pend).*(2.0./3.0)-(Ly_pend.^2.*THE_Theta_pend_D.*m_pend.*cos(THE_Phi_pend).*cos(THE_Psi_pend).^2.*cos(THE_Theta_pend).^2.*sin(THE_Theta))./6.0+Lz_pend.^2.*THE_Theta_pend_D.*m_pend.*cos(THE_Phi_pend).*cos(THE_Psi_pend).^2.*cos(THE_Theta_pend).^2.*sin(THE_Theta).*(2.0./3.0)-(Lx_pend.^2.*THE_Theta_pend_D.*m_pend.*cos(THE_Psi).*cos(THE_Theta).*cos(THE_Theta_pend).*sin(THE_Theta_pend))./6.0+(Ly_pend.^2.*THE_Psi_pend_D.*m_pend.*cos(THE_Theta).*cos(THE_Phi_pend).*cos(THE_Theta_pend).*sin(THE_Psi))./6.0+(Ly_pend.^2.*THE_Theta_pend_D.*m_pend.*cos(THE_Psi).*cos(THE_Theta).*cos(THE_Theta_pend).*sin(THE_Theta_pend))./6.0+(Lx_pend.^2.*THE_Phi_pend_D.*m_pend.*cos(THE_Theta_pend).*sin(THE_Theta).*sin(THE_Phi_pend).*sin(THE_Theta_pend))./1.2e+1-(Ly_pend.^2.*THE_Phi_pend_D.*m_pend.*cos(THE_Theta_pend).*sin(THE_Theta).*sin(THE_Phi_pend).*sin(THE_Theta_pend))./1.2e+1+(Ly_pend.^2.*THE_Theta_pend_D.*m_pend.*cos(THE_Theta).*cos(THE_Psi_pend).^2.*cos(THE_Theta_pend).^2.*sin(THE_Psi).*sin(THE_Phi_pend))./6.0-Lz_pend.^2.*THE_Theta_pend_D.*m_pend.*cos(THE_Theta).*cos(THE_Psi_pend).^2.*cos(THE_Theta_pend).^2.*sin(THE_Psi).*sin(THE_Phi_pend).*(2.0./3.0)+(Lx_pend.^2.*THE_Phi_pend_D.*m_pend.*cos(THE_Theta).*cos(THE_Phi_pend).*cos(THE_Theta_pend).*sin(THE_Psi).*sin(THE_Theta_pend))./1.2e+1-(Ly_pend.^2.*THE_Phi_pend_D.*m_pend.*cos(THE_Theta).*cos(THE_Phi_pend).*cos(THE_Theta_pend).*sin(THE_Psi).*sin(THE_Theta_pend))./1.2e+1-(Ly_pend.^2.*THE_Phi_pend_D.*m_pend.*cos(THE_Phi_pend).*cos(THE_Psi_pend).*cos(THE_Theta_pend).*sin(THE_Theta).*sin(THE_Psi_pend))./1.2e+1+(Lz_pend.^2.*THE_Phi_pend_D.*m_pend.*cos(THE_Phi_pend).*cos(THE_Psi_pend).*cos(THE_Theta_pend).*sin(THE_Theta).*sin(THE_Psi_pend))./3.0+Lz_pend.*THE_Psi_pend_D.*Tv_Z_pend.*m_pend.*cos(THE_Theta).*cos(THE_Phi_pend).*cos(THE_Psi_pend).*sin(THE_Psi)+Lz_pend.*THE_Theta_pend_D.*Tv_Z_pend.*m_pend.*cos(THE_Phi_pend).*cos(THE_Psi_pend).*cos(THE_Theta_pend).*sin(THE_Theta)-(Lz_pend.*THE_Phi_pend_D.*Tv_Z_pend.*m_pend.*cos(THE_Theta).*sin(THE_Psi).*sin(THE_Phi_pend).*sin(THE_Psi_pend))./2.0-(Lz_pend.*THE_Phi_pend_D.*Tv_Z_pend.*m_pend.*cos(THE_Psi_pend).*sin(THE_Theta).*sin(THE_Phi_pend).*sin(THE_Theta_pend))./2.0-Lz_pend.*THE_Psi_pend_D.*Tv_Z_pend.*m_pend.*cos(THE_Phi_pend).*sin(THE_Theta).*sin(THE_Psi_pend).*sin(THE_Theta_pend)-(Ly_pend.^2.*THE_Psi_pend_D.*m_pend.*cos(THE_Theta).*cos(THE_Phi_pend).*cos(THE_Psi_pend).^2.*cos(THE_Theta_pend).*sin(THE_Psi))./6.0-(Ly_pend.^2.*THE_Psi_pend_D.*m_pend.*cos(THE_Psi).*cos(THE_Theta).*cos(THE_Psi_pend).*cos(THE_Theta_pend).^2.*sin(THE_Psi_pend))./6.0-(Ly_pend.^2.*THE_Theta_pend_D.*m_pend.*cos(THE_Psi).*cos(THE_Theta).*cos(THE_Psi_pend).^2.*cos(THE_Theta_pend).*sin(THE_Theta_pend))./6.0+Lz_pend.^2.*THE_Psi_pend_D.*m_pend.*cos(THE_Theta).*cos(THE_Phi_pend).*cos(THE_Psi_pend).^2.*cos(THE_Theta_pend).*sin(THE_Psi).*(2.0./3.0)+Lz_pend.^2.*THE_Psi_pend_D.*m_pend.*cos(THE_Psi).*cos(THE_Theta).*cos(THE_Psi_pend).*cos(THE_Theta_pend).^2.*sin(THE_Psi_pend).*(2.0./3.0)+Lz_pend.^2.*THE_Theta_pend_D.*m_pend.*cos(THE_Psi).*cos(THE_Theta).*cos(THE_Psi_pend).^2.*cos(THE_Theta_pend).*sin(THE_Theta_pend).*(2.0./3.0)+(Ly_pend.^2.*THE_Phi_pend_D.*m_pend.*cos(THE_Psi_pend).^2.*cos(THE_Theta_pend).*sin(THE_Theta).*sin(THE_Phi_pend).*sin(THE_Theta_pend))./1.2e+1-(Lz_pend.^2.*THE_Phi_pend_D.*m_pend.*cos(THE_Psi_pend).^2.*cos(THE_Theta_pend).*sin(THE_Theta).*sin(THE_Phi_pend).*sin(THE_Theta_pend))./3.0+(Ly_pend.^2.*THE_Phi_pend_D.*m_pend.*cos(THE_Theta).*cos(THE_Psi_pend).*cos(THE_Theta_pend).*sin(THE_Psi).*sin(THE_Phi_pend).*sin(THE_Psi_pend))./1.2e+1+(Ly_pend.^2.*THE_Psi_pend_D.*m_pend.*cos(THE_Phi_pend).*cos(THE_Psi_pend).*cos(THE_Theta_pend).*sin(THE_Theta).*sin(THE_Psi_pend).*sin(THE_Theta_pend))./6.0-(Lz_pend.^2.*THE_Phi_pend_D.*m_pend.*cos(THE_Theta).*cos(THE_Psi_pend).*cos(THE_Theta_pend).*sin(THE_Psi).*sin(THE_Phi_pend).*sin(THE_Psi_pend))./3.0-Lz_pend.^2.*THE_Psi_pend_D.*m_pend.*cos(THE_Phi_pend).*cos(THE_Psi_pend).*cos(THE_Theta_pend).*sin(THE_Theta).*sin(THE_Psi_pend).*sin(THE_Theta_pend).*(2.0./3.0)-(Lz_pend.*THE_Phi_pend_D.*Tv_Z_pend.*m_pend.*cos(THE_Theta).*cos(THE_Phi_pend).*cos(THE_Psi_pend).*sin(THE_Psi).*sin(THE_Theta_pend))./2.0-Lz_pend.*THE_Theta_pend_D.*Tv_Z_pend.*m_pend.*cos(THE_Theta).*cos(THE_Psi_pend).*cos(THE_Theta_pend).*sin(THE_Psi).*sin(THE_Phi_pend)+Lz_pend.*THE_Psi_pend_D.*Tv_Z_pend.*m_pend.*cos(THE_Theta).*sin(THE_Psi).*sin(THE_Phi_pend).*sin(THE_Psi_pend).*sin(THE_Theta_pend)+(Ly_pend.^2.*THE_Phi_pend_D.*m_pend.*cos(THE_Theta).*cos(THE_Phi_pend).*cos(THE_Psi_pend).^2.*cos(THE_Theta_pend).*sin(THE_Psi).*sin(THE_Theta_pend))./1.2e+1-(Lz_pend.^2.*THE_Phi_pend_D.*m_pend.*cos(THE_Theta).*cos(THE_Phi_pend).*cos(THE_Psi_pend).^2.*cos(THE_Theta_pend).*sin(THE_Psi).*sin(THE_Theta_pend))./3.0-(Ly_pend.^2.*THE_Psi_pend_D.*m_pend.*cos(THE_Theta).*cos(THE_Psi_pend).*cos(THE_Theta_pend).*sin(THE_Psi).*sin(THE_Phi_pend).*sin(THE_Psi_pend).*sin(THE_Theta_pend))./6.0+Lz_pend.^2.*THE_Psi_pend_D.*m_pend.*cos(THE_Theta).*cos(THE_Psi_pend).*cos(THE_Theta_pend).*sin(THE_Psi).*sin(THE_Phi_pend).*sin(THE_Psi_pend).*sin(THE_Theta_pend).*(2.0./3.0),Lx_pend.^2.*THE_Theta_pend_D.*m_pend.*cos(THE_Psi).*sin(THE_Phi_pend).*(-1.0./6.0)+(Lx_pend.^2.*THE_Theta_pend_D.*m_pend.*cos(THE_Theta_pend).*sin(THE_Psi).*sin(THE_Theta_pend))./6.0-(Ly_pend.^2.*THE_Theta_pend_D.*m_pend.*cos(THE_Theta_pend).*sin(THE_Psi).*sin(THE_Theta_pend))./6.0+(Lx_pend.^2.*THE_Theta_pend_D.*m_pend.*cos(THE_Psi).*cos(THE_Theta_pend).^2.*sin(THE_Phi_pend))./6.0-(Ly_pend.^2.*THE_Theta_pend_D.*m_pend.*cos(THE_Psi).*cos(THE_Theta_pend).^2.*sin(THE_Phi_pend))./6.0+(Ly_pend.^2.*THE_Psi_pend_D.*m_pend.*cos(THE_Psi).*cos(THE_Phi_pend).*cos(THE_Theta_pend))./6.0-(Lz_pend.*THE_Phi_pend_D.*Tv_Z_pend.*m_pend.*cos(THE_Psi).*sin(THE_Phi_pend).*sin(THE_Psi_pend))./2.0-(Ly_pend.^2.*THE_Psi_pend_D.*m_pend.*cos(THE_Psi).*cos(THE_Phi_pend).*cos(THE_Psi_pend).^2.*cos(THE_Theta_pend))./6.0+Lz_pend.^2.*THE_Psi_pend_D.*m_pend.*cos(THE_Psi).*cos(THE_Phi_pend).*cos(THE_Psi_pend).^2.*cos(THE_Theta_pend).*(2.0./3.0)+(Ly_pend.^2.*THE_Psi_pend_D.*m_pend.*cos(THE_Psi_pend).*cos(THE_Theta_pend).^2.*sin(THE_Psi).*sin(THE_Psi_pend))./6.0+(Ly_pend.^2.*THE_Theta_pend_D.*m_pend.*cos(THE_Psi_pend).^2.*cos(THE_Theta_pend).*sin(THE_Psi).*sin(THE_Theta_pend))./6.0-Lz_pend.^2.*THE_Psi_pend_D.*m_pend.*cos(THE_Psi_pend).*cos(THE_Theta_pend).^2.*sin(THE_Psi).*sin(THE_Psi_pend).*(2.0./3.0)-Lz_pend.^2.*THE_Theta_pend_D.*m_pend.*cos(THE_Psi_pend).^2.*cos(THE_Theta_pend).*sin(THE_Psi).*sin(THE_Theta_pend).*(2.0./3.0)+(Ly_pend.^2.*THE_Theta_pend_D.*m_pend.*cos(THE_Psi).*cos(THE_Psi_pend).^2.*cos(THE_Theta_pend).^2.*sin(THE_Phi_pend))./6.0-Lz_pend.^2.*THE_Theta_pend_D.*m_pend.*cos(THE_Psi).*cos(THE_Psi_pend).^2.*cos(THE_Theta_pend).^2.*sin(THE_Phi_pend).*(2.0./3.0)+(Lx_pend.^2.*THE_Phi_pend_D.*m_pend.*cos(THE_Psi).*cos(THE_Phi_pend).*cos(THE_Theta_pend).*sin(THE_Theta_pend))./1.2e+1-(Ly_pend.^2.*THE_Phi_pend_D.*m_pend.*cos(THE_Psi).*cos(THE_Phi_pend).*cos(THE_Theta_pend).*sin(THE_Theta_pend))./1.2e+1+Lz_pend.*THE_Psi_pend_D.*Tv_Z_pend.*m_pend.*cos(THE_Psi).*cos(THE_Phi_pend).*cos(THE_Psi_pend)+(Ly_pend.^2.*THE_Phi_pend_D.*m_pend.*cos(THE_Psi).*cos(THE_Psi_pend).*cos(THE_Theta_pend).*sin(THE_Phi_pend).*sin(THE_Psi_pend))./1.2e+1-(Lz_pend.^2.*THE_Phi_pend_D.*m_pend.*cos(THE_Psi).*cos(THE_Psi_pend).*cos(THE_Theta_pend).*sin(THE_Phi_pend).*sin(THE_Psi_pend))./3.0-(Lz_pend.*THE_Phi_pend_D.*Tv_Z_pend.*m_pend.*cos(THE_Psi).*cos(THE_Phi_pend).*cos(THE_Psi_pend).*sin(THE_Theta_pend))./2.0-Lz_pend.*THE_Theta_pend_D.*Tv_Z_pend.*m_pend.*cos(THE_Psi).*cos(THE_Psi_pend).*cos(THE_Theta_pend).*sin(THE_Phi_pend)+Lz_pend.*THE_Psi_pend_D.*Tv_Z_pend.*m_pend.*cos(THE_Psi).*sin(THE_Phi_pend).*sin(THE_Psi_pend).*sin(THE_Theta_pend)+(Ly_pend.^2.*THE_Phi_pend_D.*m_pend.*cos(THE_Psi).*cos(THE_Phi_pend).*cos(THE_Psi_pend).^2.*cos(THE_Theta_pend).*sin(THE_Theta_pend))./1.2e+1-(Lz_pend.^2.*THE_Phi_pend_D.*m_pend.*cos(THE_Psi).*cos(THE_Phi_pend).*cos(THE_Psi_pend).^2.*cos(THE_Theta_pend).*sin(THE_Theta_pend))./3.0-(Ly_pend.^2.*THE_Psi_pend_D.*m_pend.*cos(THE_Psi).*cos(THE_Psi_pend).*cos(THE_Theta_pend).*sin(THE_Phi_pend).*sin(THE_Psi_pend).*sin(THE_Theta_pend))./6.0+Lz_pend.^2.*THE_Psi_pend_D.*m_pend.*cos(THE_Psi).*cos(THE_Psi_pend).*cos(THE_Theta_pend).*sin(THE_Phi_pend).*sin(THE_Psi_pend).*sin(THE_Theta_pend).*(2.0./3.0),Lx_pend.^2.*THE_Theta_pend_D.*m_pend.*cos(THE_Phi_pend).*(-1.0./6.0)-(Ly_pend.^2.*THE_Psi_pend_D.*m_pend.*cos(THE_Theta_pend).*sin(THE_Phi_pend))./6.0+(Lx_pend.^2.*THE_Theta_pend_D.*m_pend.*cos(THE_Phi_pend).*cos(THE_Theta_pend).^2)./6.0-(Ly_pend.^2.*THE_Theta_pend_D.*m_pend.*cos(THE_Phi_pend).*cos(THE_Theta_pend).^2)./6.0-(Lx_pend.^2.*THE_Phi_pend_D.*m_pend.*cos(THE_Theta_pend).*sin(THE_Phi_pend).*sin(THE_Theta_pend))./1.2e+1+(Ly_pend.^2.*THE_Phi_pend_D.*m_pend.*cos(THE_Theta_pend).*sin(THE_Phi_pend).*sin(THE_Theta_pend))./1.2e+1-(Lz_pend.*THE_Phi_pend_D.*Tv_Z_pend.*m_pend.*cos(THE_Phi_pend).*sin(THE_Psi_pend))./2.0-Lz_pend.*THE_Psi_pend_D.*Tv_Z_pend.*m_pend.*cos(THE_Psi_pend).*sin(THE_Phi_pend)+(Ly_pend.^2.*THE_Psi_pend_D.*m_pend.*cos(THE_Psi_pend).^2.*cos(THE_Theta_pend).*sin(THE_Phi_pend))./6.0-Lz_pend.^2.*THE_Psi_pend_D.*m_pend.*cos(THE_Psi_pend).^2.*cos(THE_Theta_pend).*sin(THE_Phi_pend).*(2.0./3.0)+(Ly_pend.^2.*THE_Theta_pend_D.*m_pend.*cos(THE_Phi_pend).*cos(THE_Psi_pend).^2.*cos(THE_Theta_pend).^2)./6.0-Lz_pend.^2.*THE_Theta_pend_D.*m_pend.*cos(THE_Phi_pend).*cos(THE_Psi_pend).^2.*cos(THE_Theta_pend).^2.*(2.0./3.0)+(Lz_pend.*THE_Phi_pend_D.*Tv_Z_pend.*m_pend.*cos(THE_Psi_pend).*sin(THE_Phi_pend).*sin(THE_Theta_pend))./2.0+Lz_pend.*THE_Psi_pend_D.*Tv_Z_pend.*m_pend.*cos(THE_Phi_pend).*sin(THE_Psi_pend).*sin(THE_Theta_pend)-(Ly_pend.^2.*THE_Phi_pend_D.*m_pend.*cos(THE_Psi_pend).^2.*cos(THE_Theta_pend).*sin(THE_Phi_pend).*sin(THE_Theta_pend))./1.2e+1+(Lz_pend.^2.*THE_Phi_pend_D.*m_pend.*cos(THE_Psi_pend).^2.*cos(THE_Theta_pend).*sin(THE_Phi_pend).*sin(THE_Theta_pend))./3.0+(Ly_pend.^2.*THE_Phi_pend_D.*m_pend.*cos(THE_Phi_pend).*cos(THE_Psi_pend).*cos(THE_Theta_pend).*sin(THE_Psi_pend))./1.2e+1-(Lz_pend.^2.*THE_Phi_pend_D.*m_pend.*cos(THE_Phi_pend).*cos(THE_Psi_pend).*cos(THE_Theta_pend).*sin(THE_Psi_pend))./3.0-Lz_pend.*THE_Theta_pend_D.*Tv_Z_pend.*m_pend.*cos(THE_Phi_pend).*cos(THE_Psi_pend).*cos(THE_Theta_pend)-(Ly_pend.^2.*THE_Psi_pend_D.*m_pend.*cos(THE_Phi_pend).*cos(THE_Psi_pend).*cos(THE_Theta_pend).*sin(THE_Psi_pend).*sin(THE_Theta_pend))./6.0+Lz_pend.^2.*THE_Psi_pend_D.*m_pend.*cos(THE_Phi_pend).*cos(THE_Psi_pend).*cos(THE_Theta_pend).*sin(THE_Psi_pend).*sin(THE_Theta_pend).*(2.0./3.0),Lz_pend.*m_pend.*(THE_Psi_pend_D.*cos(THE_Phi).*cos(THE_Theta).*cos(THE_Phi_pend).*cos(THE_Psi_pend).*-2.0+THE_Phi_pend_D.*cos(THE_Psi).*cos(THE_Phi_pend).*sin(THE_Phi).*sin(THE_Psi_pend)+THE_Psi_pend_D.*cos(THE_Psi).*cos(THE_Psi_pend).*sin(THE_Phi).*sin(THE_Phi_pend).*2.0+THE_Phi_pend_D.*cos(THE_Phi).*cos(THE_Theta).*sin(THE_Phi_pend).*sin(THE_Psi_pend)+THE_Phi_pend_D.*cos(THE_Phi).*cos(THE_Theta).*cos(THE_Phi_pend).*cos(THE_Psi_pend).*sin(THE_Theta_pend)+THE_Theta_pend_D.*cos(THE_Psi).*cos(THE_Phi_pend).*cos(THE_Psi_pend).*cos(THE_Theta_pend).*sin(THE_Phi).*2.0+THE_Theta_pend_D.*cos(THE_Phi).*cos(THE_Theta).*cos(THE_Psi_pend).*cos(THE_Theta_pend).*sin(THE_Phi_pend).*2.0-THE_Phi_pend_D.*cos(THE_Phi).*cos(THE_Phi_pend).*sin(THE_Psi).*sin(THE_Theta).*sin(THE_Psi_pend)-THE_Psi_pend_D.*cos(THE_Phi).*cos(THE_Psi_pend).*sin(THE_Psi).*sin(THE_Theta).*sin(THE_Phi_pend).*2.0-THE_Phi_pend_D.*cos(THE_Psi).*cos(THE_Psi_pend).*sin(THE_Phi).*sin(THE_Phi_pend).*sin(THE_Theta_pend)-THE_Psi_pend_D.*cos(THE_Psi).*cos(THE_Phi_pend).*sin(THE_Phi).*sin(THE_Psi_pend).*sin(THE_Theta_pend).*2.0-THE_Psi_pend_D.*cos(THE_Phi).*cos(THE_Theta).*sin(THE_Phi_pend).*sin(THE_Psi_pend).*sin(THE_Theta_pend).*2.0-THE_Theta_pend_D.*cos(THE_Phi).*cos(THE_Phi_pend).*cos(THE_Psi_pend).*cos(THE_Theta_pend).*sin(THE_Psi).*sin(THE_Theta).*2.0+THE_Phi_pend_D.*cos(THE_Phi).*cos(THE_Psi_pend).*sin(THE_Psi).*sin(THE_Theta).*sin(THE_Phi_pend).*sin(THE_Theta_pend)+THE_Psi_pend_D.*cos(THE_Phi).*cos(THE_Phi_pend).*sin(THE_Psi).*sin(THE_Theta).*sin(THE_Psi_pend).*sin(THE_Theta_pend).*2.0).*(-1.0./2.0),(Lz_pend.*m_pend.*(THE_Phi_pend_D.*cos(THE_Phi).*cos(THE_Psi).*cos(THE_Phi_pend).*sin(THE_Psi_pend)+THE_Psi_pend_D.*cos(THE_Phi).*cos(THE_Psi).*cos(THE_Psi_pend).*sin(THE_Phi_pend).*2.0+THE_Psi_pend_D.*cos(THE_Theta).*cos(THE_Phi_pend).*cos(THE_Psi_pend).*sin(THE_Phi).*2.0-THE_Phi_pend_D.*cos(THE_Theta).*sin(THE_Phi).*sin(THE_Phi_pend).*sin(THE_Psi_pend)+THE_Theta_pend_D.*cos(THE_Phi).*cos(THE_Psi).*cos(THE_Phi_pend).*cos(THE_Psi_pend).*cos(THE_Theta_pend).*2.0-THE_Phi_pend_D.*cos(THE_Phi).*cos(THE_Psi).*cos(THE_Psi_pend).*sin(THE_Phi_pend).*sin(THE_Theta_pend)-THE_Psi_pend_D.*cos(THE_Phi).*cos(THE_Psi).*cos(THE_Phi_pend).*sin(THE_Psi_pend).*sin(THE_Theta_pend).*2.0-THE_Phi_pend_D.*cos(THE_Theta).*cos(THE_Phi_pend).*cos(THE_Psi_pend).*sin(THE_Phi).*sin(THE_Theta_pend)-THE_Theta_pend_D.*cos(THE_Theta).*cos(THE_Psi_pend).*cos(THE_Theta_pend).*sin(THE_Phi).*sin(THE_Phi_pend).*2.0+THE_Phi_pend_D.*cos(THE_Phi_pend).*sin(THE_Phi).*sin(THE_Psi).*sin(THE_Theta).*sin(THE_Psi_pend)+THE_Psi_pend_D.*cos(THE_Psi_pend).*sin(THE_Phi).*sin(THE_Psi).*sin(THE_Theta).*sin(THE_Phi_pend).*2.0+THE_Psi_pend_D.*cos(THE_Theta).*sin(THE_Phi).*sin(THE_Phi_pend).*sin(THE_Psi_pend).*sin(THE_Theta_pend).*2.0+THE_Theta_pend_D.*cos(THE_Phi_pend).*cos(THE_Psi_pend).*cos(THE_Theta_pend).*sin(THE_Phi).*sin(THE_Psi).*sin(THE_Theta).*2.0-THE_Phi_pend_D.*cos(THE_Psi_pend).*sin(THE_Phi).*sin(THE_Psi).*sin(THE_Theta).*sin(THE_Phi_pend).*sin(THE_Theta_pend)-THE_Psi_pend_D.*cos(THE_Phi_pend).*sin(THE_Phi).*sin(THE_Psi).*sin(THE_Theta).*sin(THE_Psi_pend).*sin(THE_Theta_pend).*2.0))./2.0,(Lz_pend.*m_pend.*(THE_Phi_pend_D.*sin(THE_Theta).*sin(THE_Phi_pend).*sin(THE_Psi_pend)-THE_Psi_pend_D.*cos(THE_Phi_pend).*cos(THE_Psi_pend).*sin(THE_Theta).*2.0+THE_Phi_pend_D.*cos(THE_Theta).*cos(THE_Phi_pend).*sin(THE_Psi).*sin(THE_Psi_pend)+THE_Psi_pend_D.*cos(THE_Theta).*cos(THE_Psi_pend).*sin(THE_Psi).*sin(THE_Phi_pend).*2.0+THE_Phi_pend_D.*cos(THE_Phi_pend).*cos(THE_Psi_pend).*sin(THE_Theta).*sin(THE_Theta_pend)+THE_Theta_pend_D.*cos(THE_Psi_pend).*cos(THE_Theta_pend).*sin(THE_Theta).*sin(THE_Phi_pend).*2.0-THE_Psi_pend_D.*sin(THE_Theta).*sin(THE_Phi_pend).*sin(THE_Psi_pend).*sin(THE_Theta_pend).*2.0+THE_Theta_pend_D.*cos(THE_Theta).*cos(THE_Phi_pend).*cos(THE_Psi_pend).*cos(THE_Theta_pend).*sin(THE_Psi).*2.0-THE_Phi_pend_D.*cos(THE_Theta).*cos(THE_Psi_pend).*sin(THE_Psi).*sin(THE_Phi_pend).*sin(THE_Theta_pend)-THE_Psi_pend_D.*cos(THE_Theta).*cos(THE_Phi_pend).*sin(THE_Psi).*sin(THE_Psi_pend).*sin(THE_Theta_pend).*2.0))./2.0,m_pend.*cos(THE_Theta_pend).*(Lx_pend.^2.*THE_Theta_pend_D.*sin(THE_Theta_pend)-Ly_pend.^2.*THE_Theta_pend_D.*sin(THE_Theta_pend)+Ly_pend.^2.*THE_Theta_pend_D.*cos(THE_Psi_pend).^2.*sin(THE_Theta_pend)-Lz_pend.^2.*THE_Theta_pend_D.*cos(THE_Psi_pend).^2.*sin(THE_Theta_pend).*4.0+Ly_pend.^2.*THE_Psi_pend_D.*cos(THE_Psi_pend).*cos(THE_Theta_pend).*sin(THE_Psi_pend)-Lz_pend.^2.*THE_Psi_pend_D.*cos(THE_Psi_pend).*cos(THE_Theta_pend).*sin(THE_Psi_pend).*4.0).*(-1.0./6.0),(m_pend.*cos(THE_Theta_pend).*(Ly_pend.^2.*THE_Psi_pend_D.*2.0+Lx_pend.^2.*THE_Phi_pend_D.*sin(THE_Theta_pend)-Ly_pend.^2.*THE_Phi_pend_D.*sin(THE_Theta_pend)-Ly_pend.^2.*THE_Psi_pend_D.*cos(THE_Psi_pend).^2.*2.0+Lz_pend.^2.*THE_Psi_pend_D.*cos(THE_Psi_pend).^2.*8.0+Ly_pend.^2.*THE_Phi_pend_D.*cos(THE_Psi_pend).^2.*sin(THE_Theta_pend)-Lz_pend.^2.*THE_Phi_pend_D.*cos(THE_Psi_pend).^2.*sin(THE_Theta_pend).*4.0))./1.2e+1,m_pend.*cos(THE_Theta_pend).*(Ly_pend.^2.*THE_Theta_pend_D.*2.0-Ly_pend.^2.*THE_Theta_pend_D.*cos(THE_Psi_pend).^2.*2.0+Lz_pend.^2.*THE_Theta_pend_D.*cos(THE_Psi_pend).^2.*8.0-Ly_pend.^2.*THE_Phi_pend_D.*cos(THE_Psi_pend).*cos(THE_Theta_pend).*sin(THE_Psi_pend)+Lz_pend.^2.*THE_Phi_pend_D.*cos(THE_Psi_pend).*cos(THE_Theta_pend).*sin(THE_Psi_pend).*4.0).*(-1.0./1.2e+1),Lz_pend.^2.*THE_Psi_pend_D.*m_pend.*cos(THE_Phi_pend).*sin(THE_Theta).*sin(THE_Theta_pend).*(2.0./3.0)-Lz_pend.^2.*THE_Psi_pend_D.*m_pend.*cos(THE_Psi).*cos(THE_Theta).*cos(THE_Theta_pend).*(2.0./3.0)-(Ly_pend.^2.*THE_Psi_pend_D.*m_pend.*cos(THE_Psi).*cos(THE_Theta).*cos(THE_Psi_pend).^2.*cos(THE_Theta_pend))./6.0+Lz_pend.^2.*THE_Psi_pend_D.*m_pend.*cos(THE_Psi).*cos(THE_Theta).*cos(THE_Psi_pend).^2.*cos(THE_Theta_pend).*(2.0./3.0)+(Ly_pend.^2.*THE_Psi_pend_D.*m_pend.*cos(THE_Phi_pend).*cos(THE_Psi_pend).^2.*sin(THE_Theta).*sin(THE_Theta_pend))./6.0-Lz_pend.^2.*THE_Psi_pend_D.*m_pend.*cos(THE_Phi_pend).*cos(THE_Psi_pend).^2.*sin(THE_Theta).*sin(THE_Theta_pend).*(2.0./3.0)+(Ly_pend.^2.*THE_Psi_pend_D.*m_pend.*cos(THE_Psi_pend).*sin(THE_Theta).*sin(THE_Phi_pend).*sin(THE_Psi_pend))./6.0-Lz_pend.^2.*THE_Psi_pend_D.*m_pend.*cos(THE_Theta).*sin(THE_Psi).*sin(THE_Phi_pend).*sin(THE_Theta_pend).*(2.0./3.0)-Lz_pend.^2.*THE_Psi_pend_D.*m_pend.*cos(THE_Psi_pend).*sin(THE_Theta).*sin(THE_Phi_pend).*sin(THE_Psi_pend).*(2.0./3.0)+(Ly_pend.^2.*THE_Psi_pend_D.*m_pend.*cos(THE_Theta).*cos(THE_Phi_pend).*cos(THE_Psi_pend).*sin(THE_Psi).*sin(THE_Psi_pend))./6.0+(Ly_pend.^2.*THE_Theta_pend_D.*m_pend.*cos(THE_Psi).*cos(THE_Theta).*cos(THE_Psi_pend).*sin(THE_Psi_pend).*sin(THE_Theta_pend))./1.2e+1+(Ly_pend.^2.*THE_Theta_pend_D.*m_pend.*cos(THE_Phi_pend).*cos(THE_Psi_pend).*cos(THE_Theta_pend).*sin(THE_Theta).*sin(THE_Psi_pend))./1.2e+1-Lz_pend.^2.*THE_Psi_pend_D.*m_pend.*cos(THE_Theta).*cos(THE_Phi_pend).*cos(THE_Psi_pend).*sin(THE_Psi).*sin(THE_Psi_pend).*(2.0./3.0)-(Lz_pend.^2.*THE_Theta_pend_D.*m_pend.*cos(THE_Psi).*cos(THE_Theta).*cos(THE_Psi_pend).*sin(THE_Psi_pend).*sin(THE_Theta_pend))./3.0-(Lz_pend.^2.*THE_Theta_pend_D.*m_pend.*cos(THE_Phi_pend).*cos(THE_Psi_pend).*cos(THE_Theta_pend).*sin(THE_Theta).*sin(THE_Psi_pend))./3.0-Lz_pend.*THE_Psi_pend_D.*Tv_Z_pend.*m_pend.*cos(THE_Theta_pend).*sin(THE_Theta).*sin(THE_Phi_pend).*sin(THE_Psi_pend)-(Lz_pend.*THE_Theta_pend_D.*Tv_Z_pend.*m_pend.*cos(THE_Psi_pend).*sin(THE_Theta).*sin(THE_Phi_pend).*sin(THE_Theta_pend))./2.0-(Ly_pend.^2.*THE_Psi_pend_D.*m_pend.*cos(THE_Theta).*cos(THE_Psi_pend).^2.*sin(THE_Psi).*sin(THE_Phi_pend).*sin(THE_Theta_pend))./6.0+Lz_pend.^2.*THE_Psi_pend_D.*m_pend.*cos(THE_Theta).*cos(THE_Psi_pend).^2.*sin(THE_Psi).*sin(THE_Phi_pend).*sin(THE_Theta_pend).*(2.0./3.0)-(Ly_pend.^2.*THE_Theta_pend_D.*m_pend.*cos(THE_Theta).*cos(THE_Psi_pend).*cos(THE_Theta_pend).*sin(THE_Psi).*sin(THE_Phi_pend).*sin(THE_Psi_pend))./1.2e+1+(Lz_pend.^2.*THE_Theta_pend_D.*m_pend.*cos(THE_Theta).*cos(THE_Psi_pend).*cos(THE_Theta_pend).*sin(THE_Psi).*sin(THE_Phi_pend).*sin(THE_Psi_pend))./3.0-Lz_pend.*THE_Psi_pend_D.*Tv_Z_pend.*m_pend.*cos(THE_Theta).*cos(THE_Phi_pend).*cos(THE_Theta_pend).*sin(THE_Psi).*sin(THE_Psi_pend)-(Lz_pend.*THE_Theta_pend_D.*Tv_Z_pend.*m_pend.*cos(THE_Theta).*cos(THE_Phi_pend).*cos(THE_Psi_pend).*sin(THE_Psi).*sin(THE_Theta_pend))./2.0,Lz_pend.^2.*THE_Psi_pend_D.*m_pend.*cos(THE_Theta_pend).*sin(THE_Psi).*(2.0./3.0)-Lz_pend.^2.*THE_Psi_pend_D.*m_pend.*cos(THE_Psi).*sin(THE_Phi_pend).*sin(THE_Theta_pend).*(2.0./3.0)+(Ly_pend.^2.*THE_Psi_pend_D.*m_pend.*cos(THE_Psi_pend).^2.*cos(THE_Theta_pend).*sin(THE_Psi))./6.0-Lz_pend.^2.*THE_Psi_pend_D.*m_pend.*cos(THE_Psi_pend).^2.*cos(THE_Theta_pend).*sin(THE_Psi).*(2.0./3.0)-(Ly_pend.^2.*THE_Psi_pend_D.*m_pend.*cos(THE_Psi).*cos(THE_Psi_pend).^2.*sin(THE_Phi_pend).*sin(THE_Theta_pend))./6.0+Lz_pend.^2.*THE_Psi_pend_D.*m_pend.*cos(THE_Psi).*cos(THE_Psi_pend).^2.*sin(THE_Phi_pend).*sin(THE_Theta_pend).*(2.0./3.0)+(Ly_pend.^2.*THE_Psi_pend_D.*m_pend.*cos(THE_Psi).*cos(THE_Phi_pend).*cos(THE_Psi_pend).*sin(THE_Psi_pend))./6.0-Lz_pend.^2.*THE_Psi_pend_D.*m_pend.*cos(THE_Psi).*cos(THE_Phi_pend).*cos(THE_Psi_pend).*sin(THE_Psi_pend).*(2.0./3.0)-(Ly_pend.^2.*THE_Theta_pend_D.*m_pend.*cos(THE_Psi_pend).*sin(THE_Psi).*sin(THE_Psi_pend).*sin(THE_Theta_pend))./1.2e+1+(Lz_pend.^2.*THE_Theta_pend_D.*m_pend.*cos(THE_Psi_pend).*sin(THE_Psi).*sin(THE_Psi_pend).*sin(THE_Theta_pend))./3.0-(Ly_pend.^2.*THE_Theta_pend_D.*m_pend.*cos(THE_Psi).*cos(THE_Psi_pend).*cos(THE_Theta_pend).*sin(THE_Phi_pend).*sin(THE_Psi_pend))./1.2e+1+(Lz_pend.^2.*THE_Theta_pend_D.*m_pend.*cos(THE_Psi).*cos(THE_Psi_pend).*cos(THE_Theta_pend).*sin(THE_Phi_pend).*sin(THE_Psi_pend))./3.0-Lz_pend.*THE_Psi_pend_D.*Tv_Z_pend.*m_pend.*cos(THE_Psi).*cos(THE_Phi_pend).*cos(THE_Theta_pend).*sin(THE_Psi_pend)-(Lz_pend.*THE_Theta_pend_D.*Tv_Z_pend.*m_pend.*cos(THE_Psi).*cos(THE_Phi_pend).*cos(THE_Psi_pend).*sin(THE_Theta_pend))./2.0,Lz_pend.^2.*THE_Psi_pend_D.*m_pend.*cos(THE_Phi_pend).*sin(THE_Theta_pend).*(-2.0./3.0)-(Ly_pend.^2.*THE_Psi_pend_D.*m_pend.*cos(THE_Psi_pend).*sin(THE_Phi_pend).*sin(THE_Psi_pend))./6.0+Lz_pend.^2.*THE_Psi_pend_D.*m_pend.*cos(THE_Psi_pend).*sin(THE_Phi_pend).*sin(THE_Psi_pend).*(2.0./3.0)-(Ly_pend.^2.*THE_Psi_pend_D.*m_pend.*cos(THE_Phi_pend).*cos(THE_Psi_pend).^2.*sin(THE_Theta_pend))./6.0+Lz_pend.^2.*THE_Psi_pend_D.*m_pend.*cos(THE_Phi_pend).*cos(THE_Psi_pend).^2.*sin(THE_Theta_pend).*(2.0./3.0)+Lz_pend.*THE_Psi_pend_D.*Tv_Z_pend.*m_pend.*cos(THE_Theta_pend).*sin(THE_Phi_pend).*sin(THE_Psi_pend)+(Lz_pend.*THE_Theta_pend_D.*Tv_Z_pend.*m_pend.*cos(THE_Psi_pend).*sin(THE_Phi_pend).*sin(THE_Theta_pend))./2.0-(Ly_pend.^2.*THE_Theta_pend_D.*m_pend.*cos(THE_Phi_pend).*cos(THE_Psi_pend).*cos(THE_Theta_pend).*sin(THE_Psi_pend))./1.2e+1+(Lz_pend.^2.*THE_Theta_pend_D.*m_pend.*cos(THE_Phi_pend).*cos(THE_Psi_pend).*cos(THE_Theta_pend).*sin(THE_Psi_pend))./3.0,Lz_pend.*m_pend.*(THE_Theta_pend_D.*cos(THE_Psi_pend).*cos(THE_Theta_pend).*sin(THE_Phi).*sin(THE_Psi)-THE_Psi_pend_D.*sin(THE_Phi).*sin(THE_Psi).*sin(THE_Psi_pend).*sin(THE_Theta_pend).*2.0+THE_Theta_pend_D.*cos(THE_Phi).*cos(THE_Psi).*cos(THE_Psi_pend).*cos(THE_Theta_pend).*sin(THE_Theta)+THE_Psi_pend_D.*cos(THE_Phi).*cos(THE_Theta).*cos(THE_Phi_pend).*cos(THE_Theta_pend).*sin(THE_Psi_pend).*2.0+THE_Theta_pend_D.*cos(THE_Phi).*cos(THE_Theta).*cos(THE_Phi_pend).*cos(THE_Psi_pend).*sin(THE_Theta_pend)-THE_Psi_pend_D.*cos(THE_Phi).*cos(THE_Psi).*sin(THE_Theta).*sin(THE_Psi_pend).*sin(THE_Theta_pend).*2.0-THE_Psi_pend_D.*cos(THE_Psi).*cos(THE_Theta_pend).*sin(THE_Phi).*sin(THE_Phi_pend).*sin(THE_Psi_pend).*2.0-THE_Theta_pend_D.*cos(THE_Psi).*cos(THE_Psi_pend).*sin(THE_Phi).*sin(THE_Phi_pend).*sin(THE_Theta_pend)+THE_Psi_pend_D.*cos(THE_Phi).*cos(THE_Theta_pend).*sin(THE_Psi).*sin(THE_Theta).*sin(THE_Phi_pend).*sin(THE_Psi_pend).*2.0+THE_Theta_pend_D.*cos(THE_Phi).*cos(THE_Psi_pend).*sin(THE_Psi).*sin(THE_Theta).*sin(THE_Phi_pend).*sin(THE_Theta_pend)).*(-1.0./2.0),Lz_pend.*m_pend.*(-THE_Theta_pend_D.*cos(THE_Phi).*cos(THE_Psi_pend).*cos(THE_Theta_pend).*sin(THE_Psi)+THE_Psi_pend_D.*cos(THE_Phi).*sin(THE_Psi).*sin(THE_Psi_pend).*sin(THE_Theta_pend).*2.0+THE_Theta_pend_D.*cos(THE_Psi).*cos(THE_Psi_pend).*cos(THE_Theta_pend).*sin(THE_Phi).*sin(THE_Theta)+THE_Psi_pend_D.*cos(THE_Phi).*cos(THE_Psi).*cos(THE_Theta_pend).*sin(THE_Phi_pend).*sin(THE_Psi_pend).*2.0+THE_Psi_pend_D.*cos(THE_Theta).*cos(THE_Phi_pend).*cos(THE_Theta_pend).*sin(THE_Phi).*sin(THE_Psi_pend).*2.0+THE_Theta_pend_D.*cos(THE_Phi).*cos(THE_Psi).*cos(THE_Psi_pend).*sin(THE_Phi_pend).*sin(THE_Theta_pend)+THE_Theta_pend_D.*cos(THE_Theta).*cos(THE_Phi_pend).*cos(THE_Psi_pend).*sin(THE_Phi).*sin(THE_Theta_pend)-THE_Psi_pend_D.*cos(THE_Psi).*sin(THE_Phi).*sin(THE_Theta).*sin(THE_Psi_pend).*sin(THE_Theta_pend).*2.0+THE_Psi_pend_D.*cos(THE_Theta_pend).*sin(THE_Phi).*sin(THE_Psi).*sin(THE_Theta).*sin(THE_Phi_pend).*sin(THE_Psi_pend).*2.0+THE_Theta_pend_D.*cos(THE_Psi_pend).*sin(THE_Phi).*sin(THE_Psi).*sin(THE_Theta).*sin(THE_Phi_pend).*sin(THE_Theta_pend)).*(-1.0./2.0),Lz_pend.*m_pend.*(THE_Theta_pend_D.*cos(THE_Psi).*cos(THE_Theta).*cos(THE_Psi_pend).*cos(THE_Theta_pend)-THE_Psi_pend_D.*cos(THE_Psi).*cos(THE_Theta).*sin(THE_Psi_pend).*sin(THE_Theta_pend).*2.0-THE_Psi_pend_D.*cos(THE_Phi_pend).*cos(THE_Theta_pend).*sin(THE_Theta).*sin(THE_Psi_pend).*2.0-THE_Theta_pend_D.*cos(THE_Phi_pend).*cos(THE_Psi_pend).*sin(THE_Theta).*sin(THE_Theta_pend)+THE_Psi_pend_D.*cos(THE_Theta).*cos(THE_Theta_pend).*sin(THE_Psi).*sin(THE_Phi_pend).*sin(THE_Psi_pend).*2.0+THE_Theta_pend_D.*cos(THE_Theta).*cos(THE_Psi_pend).*sin(THE_Psi).*sin(THE_Phi_pend).*sin(THE_Theta_pend)).*(-1.0./2.0),m_pend.*(Lz_pend.^2.*THE_Psi_pend_D.*cos(THE_Theta_pend).*8.0+Ly_pend.^2.*THE_Psi_pend_D.*cos(THE_Psi_pend).^2.*cos(THE_Theta_pend).*2.0-Lz_pend.^2.*THE_Psi_pend_D.*cos(THE_Psi_pend).^2.*cos(THE_Theta_pend).*8.0-Ly_pend.^2.*THE_Theta_pend_D.*cos(THE_Psi_pend).*sin(THE_Psi_pend).*sin(THE_Theta_pend)+Lz_pend.^2.*THE_Theta_pend_D.*cos(THE_Psi_pend).*sin(THE_Psi_pend).*sin(THE_Theta_pend).*4.0).*(-1.0./1.2e+1),(THE_Psi_pend_D.*m_pend.*sin(THE_Psi_pend.*2.0).*(Ly_pend.^2-Lz_pend.^2.*4.0))./1.2e+1,THE_Theta_pend_D.*m_pend.*sin(THE_Psi_pend.*2.0).*(Ly_pend.^2-Lz_pend.^2.*4.0).*(-1.0./2.4e+1),Lz_pend.*THE_Psi_pend_D.*Tv_Z_pend.*m_pend.*(-cos(THE_Phi_pend).*sin(THE_Theta).*sin(THE_Psi_pend)+cos(THE_Theta).*sin(THE_Psi).*sin(THE_Phi_pend).*sin(THE_Psi_pend)+cos(THE_Psi_pend).*sin(THE_Theta).*sin(THE_Phi_pend).*sin(THE_Theta_pend)+cos(THE_Theta).*cos(THE_Phi_pend).*cos(THE_Psi_pend).*sin(THE_Psi).*sin(THE_Theta_pend)).*(-1.0./2.0),Lz_pend.*THE_Psi_pend_D.*Tv_Z_pend.*m_pend.*cos(THE_Psi).*(sin(THE_Phi_pend).*sin(THE_Psi_pend)+cos(THE_Phi_pend).*cos(THE_Psi_pend).*sin(THE_Theta_pend)).*(-1.0./2.0),Lz_pend.*THE_Psi_pend_D.*Tv_Z_pend.*m_pend.*(cos(THE_Phi_pend).*sin(THE_Psi_pend)-cos(THE_Psi_pend).*sin(THE_Phi_pend).*sin(THE_Theta_pend)).*(-1.0./2.0),Lz_pend.*THE_Psi_pend_D.*m_pend.*(cos(THE_Psi).*cos(THE_Phi_pend).*sin(THE_Phi).*sin(THE_Psi_pend)+cos(THE_Phi).*cos(THE_Theta).*sin(THE_Phi_pend).*sin(THE_Psi_pend)+cos(THE_Psi_pend).*cos(THE_Theta_pend).*sin(THE_Phi).*sin(THE_Psi)+cos(THE_Phi).*cos(THE_Psi).*cos(THE_Psi_pend).*cos(THE_Theta_pend).*sin(THE_Theta)+cos(THE_Phi).*cos(THE_Theta).*cos(THE_Phi_pend).*cos(THE_Psi_pend).*sin(THE_Theta_pend)-cos(THE_Phi).*cos(THE_Phi_pend).*sin(THE_Psi).*sin(THE_Theta).*sin(THE_Psi_pend)-cos(THE_Psi).*cos(THE_Psi_pend).*sin(THE_Phi).*sin(THE_Phi_pend).*sin(THE_Theta_pend)+cos(THE_Phi).*cos(THE_Psi_pend).*sin(THE_Psi).*sin(THE_Theta).*sin(THE_Phi_pend).*sin(THE_Theta_pend)).*(-1.0./2.0),Lz_pend.*THE_Psi_pend_D.*m_pend.*(-cos(THE_Phi).*cos(THE_Psi).*cos(THE_Phi_pend).*sin(THE_Psi_pend)-cos(THE_Phi).*cos(THE_Psi_pend).*cos(THE_Theta_pend).*sin(THE_Psi)+cos(THE_Theta).*sin(THE_Phi).*sin(THE_Phi_pend).*sin(THE_Psi_pend)+cos(THE_Psi).*cos(THE_Psi_pend).*cos(THE_Theta_pend).*sin(THE_Phi).*sin(THE_Theta)+cos(THE_Phi).*cos(THE_Psi).*cos(THE_Psi_pend).*sin(THE_Phi_pend).*sin(THE_Theta_pend)+cos(THE_Theta).*cos(THE_Phi_pend).*cos(THE_Psi_pend).*sin(THE_Phi).*sin(THE_Theta_pend)-cos(THE_Phi_pend).*sin(THE_Phi).*sin(THE_Psi).*sin(THE_Theta).*sin(THE_Psi_pend)+cos(THE_Psi_pend).*sin(THE_Phi).*sin(THE_Psi).*sin(THE_Theta).*sin(THE_Phi_pend).*sin(THE_Theta_pend)).*(-1.0./2.0),(Lz_pend.*THE_Psi_pend_D.*m_pend.*(sin(THE_Theta).*sin(THE_Phi_pend).*sin(THE_Psi_pend)-cos(THE_Psi).*cos(THE_Theta).*cos(THE_Psi_pend).*cos(THE_Theta_pend)+cos(THE_Theta).*cos(THE_Phi_pend).*sin(THE_Psi).*sin(THE_Psi_pend)+cos(THE_Phi_pend).*cos(THE_Psi_pend).*sin(THE_Theta).*sin(THE_Theta_pend)-cos(THE_Theta).*cos(THE_Psi_pend).*sin(THE_Psi).*sin(THE_Phi_pend).*sin(THE_Theta_pend)))./2.0,0.0,0.0,0.0],[9,9]);
end
if nargout > 2
    K = reshape([0.0,0.0,0.0,0.0,0.0,0.0,0.0,0.0,0.0,0.0,0.0,0.0,0.0,0.0,0.0,0.0,0.0,0.0,0.0,0.0,0.0,0.0,0.0,0.0,0.0,0.0,0.0,0.0,0.0,0.0,0.0,0.0,0.0,0.0,0.0,0.0,0.0,0.0,0.0,0.0,0.0,0.0,0.0,0.0,0.0,0.0,0.0,0.0,0.0,0.0,0.0,0.0,0.0,0.0,0.0,0.0,0.0,0.0,0.0,0.0,0.0,0.0,0.0,0.0,0.0,0.0,0.0,0.0,0.0,0.0,0.0,0.0,0.0,0.0,0.0,0.0,0.0,0.0,0.0,0.0,0.0],[9,9]);
end
if nargout > 3
    G = [0.0;-Tv_Z_pend.*g.*m_pend.*cos(THE_Psi).*sin(THE_Theta)-cg_to_mot_H.*g.*mprop.*cos(THE_Psi).*sin(THE_Theta).*4.0-(Lz_pend.*g.*m_pend.*cos(THE_Theta).*sin(THE_Phi_pend).*sin(THE_Psi_pend))./2.0-(Lz_pend.*g.*m_pend.*cos(THE_Psi).*cos(THE_Psi_pend).*cos(THE_Theta_pend).*sin(THE_Theta))./2.0-(Lz_pend.*g.*m_pend.*cos(THE_Theta).*cos(THE_Phi_pend).*cos(THE_Psi_pend).*sin(THE_Theta_pend))./2.0+(Lz_pend.*g.*m_pend.*cos(THE_Phi_pend).*sin(THE_Psi).*sin(THE_Theta).*sin(THE_Psi_pend))./2.0-(Lz_pend.*g.*m_pend.*cos(THE_Psi_pend).*sin(THE_Psi).*sin(THE_Theta).*sin(THE_Phi_pend).*sin(THE_Theta_pend))./2.0;g.*cos(THE_Theta).*(Tv_Z_pend.*m_pend.*sin(THE_Psi).*2.0+cg_to_mot_H.*mprop.*sin(THE_Psi).*8.0+Lz_pend.*m_pend.*cos(THE_Psi).*cos(THE_Phi_pend).*sin(THE_Psi_pend)+Lz_pend.*m_pend.*cos(THE_Psi_pend).*cos(THE_Theta_pend).*sin(THE_Psi)-Lz_pend.*m_pend.*cos(THE_Psi).*cos(THE_Psi_pend).*sin(THE_Phi_pend).*sin(THE_Theta_pend)).*(-1.0./2.0);0.0;0.0;g.*(m+m_pend+mprop.*4.0);(Lz_pend.*g.*m_pend.*(-cos(THE_Phi_pend).*sin(THE_Theta).*sin(THE_Psi_pend)+cos(THE_Theta).*sin(THE_Psi).*sin(THE_Phi_pend).*sin(THE_Psi_pend)+cos(THE_Psi_pend).*sin(THE_Theta).*sin(THE_Phi_pend).*sin(THE_Theta_pend)+cos(THE_Theta).*cos(THE_Phi_pend).*cos(THE_Psi_pend).*sin(THE_Psi).*sin(THE_Theta_pend)))./2.0;Lz_pend.*g.*m_pend.*cos(THE_Psi_pend).*(cos(THE_Psi).*cos(THE_Theta).*sin(THE_Theta_pend)+cos(THE_Phi_pend).*cos(THE_Theta_pend).*sin(THE_Theta)-cos(THE_Theta).*cos(THE_Theta_pend).*sin(THE_Psi).*sin(THE_Phi_pend)).*(-1.0./2.0);Lz_pend.*g.*m_pend.*(cos(THE_Psi_pend).*sin(THE_Theta).*sin(THE_Phi_pend)+cos(THE_Theta).*cos(THE_Phi_pend).*cos(THE_Psi_pend).*sin(THE_Psi)+cos(THE_Psi).*cos(THE_Theta).*cos(THE_Theta_pend).*sin(THE_Psi_pend)-cos(THE_Phi_pend).*sin(THE_Theta).*sin(THE_Psi_pend).*sin(THE_Theta_pend)+cos(THE_Theta).*sin(THE_Psi).*sin(THE_Phi_pend).*sin(THE_Psi_pend).*sin(THE_Theta_pend)).*(-1.0./2.0)];
end
if nargout > 4
    Q = [Mbz_1.*cos(THE_Psi).*cos(THE_Theta)+Mbz_2.*cos(THE_Psi).*cos(THE_Theta)+Mbz_3.*cos(THE_Psi).*cos(THE_Theta)+Mbz_4.*cos(THE_Psi).*cos(THE_Theta)-Tbz_2.*cg_to_mot_L.*sin(THE_Theta)+Tbz_4.*cg_to_mot_L.*sin(THE_Theta)-Tbz_1.*cg_to_mot_L.*cos(THE_Theta).*sin(THE_Psi)+Tbz_3.*cg_to_mot_L.*cos(THE_Theta).*sin(THE_Psi);-Mbz_1.*sin(THE_Psi)-Mbz_2.*sin(THE_Psi)-Mbz_3.*sin(THE_Psi)-Mbz_4.*sin(THE_Psi)-Tbz_1.*cg_to_mot_L.*cos(THE_Psi)+Tbz_3.*cg_to_mot_L.*cos(THE_Psi);cg_to_mot_L.*(Tbz_2-Tbz_4);(sin(THE_Phi).*sin(THE_Psi)+cos(THE_Phi).*cos(THE_Psi).*sin(THE_Theta)).*(Tbz_1+Tbz_2+Tbz_3+Tbz_4);-(cos(THE_Phi).*sin(THE_Psi)-cos(THE_Psi).*sin(THE_Phi).*sin(THE_Theta)).*(Tbz_1+Tbz_2+Tbz_3+Tbz_4);cos(THE_Psi).*cos(THE_Theta).*(Tbz_1+Tbz_2+Tbz_3+Tbz_4);0.0;0.0;0.0];
end
